simulink model "simulink_slipsl"  (R2022b)
settings: Solver=ode45  StartTime=0.0  StopTime=Tf  FixedStep=1e-3  RelTol=1e-11  AbsTol=1e-11
values from neighbouring files (symbols this model uses):
  flag_dist = [0; 30; 30]    [main.m]    (also in main_slip_w_sw_leg.m = 0)
  gains = [gain.K_p; gain.K_d; gain.K_p_sw; gain.K_d_sw; gain.K_p_ds; gain.K_d_ds; gain.K_v_ds]    [main.m]    (also in main_slip_w_sw_leg.m)
  init_cond = [x_M_init; y_M_init; theta_init; r_init; x_CoM_init; y_CoM_init; dx_M_init; dy_M_init; dtheta_init; dr_init; dx_CoM_init; dy_CoM_init]    [main.m]    (also in main_slip_w_sw_leg.m)
  init_f_record = 0    [main.m]    (also in main_slip_w_sw_leg.m)
  init_flag = [1; dc.col_param.foot; -dc.col_param.footPlus; x_M_init; x_CoM_ss_init; flag_ref_ob]    [main.m]    (also in main_slip_w_sw_leg.m = [1; dc.col_param.foot; -dc.col_param.footPlus; x_M_init; x_C)
  param = [L0_ss; k0_ss; m_M; m_swLeg; m_swFoot; I_swLeg; I_swFoot; L_thigh; k_swFoot; k_swLeg; theta_s0; r_s0; g; L0_ds; k0_ds; bound_cst]    [main.m]    (also in main_slip_w_sw_leg.m = [L0_ss; k0_ss; m_M; m_swLeg; m_swFoot; I_swLeg; I_swFoot; L_)
  ref_star_ds = [ref_star.ds.x_CoM_star,      ref_star.ds.y_CoM_star, ref_star.ds.dx_CoM_star,      ref_star.ds.del_y_CoM_star, ref_star.ds.del_dx_CoM_star,      ref_star.ds.del2_y_CoM_star]    [main.m]    (also in main_slip_w_sw_leg.m)
  ref_star_ss = [ref_star.ss.x_M_star,      ref_star.ss.y_M_star, ref_star.ss.x_swFoot_star, ref_star.ss.y_swFoot_star,      ref_star.ss.del_y_M_star, ref_star.ss.del_x_swFoot_star, ref_star.ss.del_y_swFoot_star,      ref_star.ss.del2_y_M_star, ref_star.ss.del2_x_swFoot_star, ref_star.ss.del2_y_swFoot_star,      ref_star.ss.x_CoM_star]    [main.m]    (also in main_slip_w_sw_leg.m)
  sample_time = 0.001    [main.m]    (also in main_slip_w_sw_leg.m)
libraries: simulink x1
(part 2 of 2)

== matlab function simulink_slipsl/Triggered Subsystem/SLIP-SL controller ==
  data: X input; U output; flag input; ref_star_ss input; ref_star_ds input; gains input; param input; ref_output_ss output; ref_output_ds output; det_A_ss output; det_A_ds output
function [U, ref_output_ss, ref_output_ds, det_A_ss, det_A_ds] = fcn(X, flag, ref_star_ss, ref_star_ds, gains, param)

% ----------- parameters ----------------------
L0_ss = param(1); % [m]
k0_ss = param(2); % nominal leg stiffness [N/m]
m_M = param(3); % hip mass [kg]
m_swLeg = param(4); % [kg]
m_swFoot = param(5); % [kg]
I_swLeg = param(6); %
I_swFoot = param(7); %
L_thigh = param(8); % [m]
k_swFoot = param(9); %
k_swLeg = param(10); %
theta0 = param(11); %[rad]
r0 = param(12); % [m]
gravi = param(13); % gravitational acc

L0_ds = param(14); % [m] free length of the springs in the DS
k0_ds = param(15); % [N/m] stiffness of the springs in the DS

% ----------- flags ----------------------
f_stance = flag(1); % indicates which stance phase it is
foot = flag(2); % location of the stance foot
foot_prev = flag(3) - foot; % previous location of the stance foot
x_M_LO = flag(4); % x_M @LO
x_CoM_LO = flag(5); % x_CoM @LO

% ----------- states ----------------------
x_M = X(1) - foot; % x position of main mass in SS
y_M = X(2); % z position of main mass in SS
theta = X(3); % angle of the swing leg when in SS
r = X(4); % distance of the foot from the knee on SS
x_CoM = X(5) - foot; % x position of the CoM
y_CoM = X(6);

dx_M = X(7); % x velocity of main mass in SS
dy_M = X(8); % z velocity of main mass in SS
dtheta = X(9);
dr = X(10);
dx_CoM = X(11);
dy_CoM = X(12);

q = [x_M; y_M; theta; r; x_CoM; y_CoM];
dq = [dx_M; dy_M; dtheta; dr; dx_CoM; dy_CoM];

%---------- controller -----------------------------

% SS inputs
u1 = 0; % input for stance leg spring
u2 = 0; % input for swing leg torsional spring
u3 = 0; % input for swing foot spring
% DS inputs
u4 = 0; % input for stance leg spring
u5 = 0; % input for swing leg spring

% Controller Gains
K_p = gains(1);
K_d = gains(2);

K_p_sw = gains(3);
K_d_sw = gains(4);

K_p_ds = gains(5);
K_d_ds = gains(6);
K_v_ds = gains(7); % 5 in visser 2012

% for debugging
ref_output_ss = [0; 0; 0];
ref_output_ds = [0;0];
det_A_ss = -1;
det_A_ds = 0;

x_CoM_star_ds = ref_star_ds(:,1);

if f_stance == 1
    % if the system is in single stance phase

    x_CoM_star_ss = ref_star_ss(:,11);

    % updating the x_CoM_star_ss
    x_CoM_des_TD = ref_star_ss(end,11);
    x_CoM_star_ss = x_CoM_star_ss.*((x_CoM_des_TD - x_CoM_LO)/(ref_star_ss(end,11) - ref_star_ss(1,11))) + (x_CoM_LO - ref_star_ss(1,11))/2;

    % calculating x_CoM when for SS phase
    x_swLeg = x_M + (L_thigh/2)*cos(theta);
    x_swFoot = x_M + (L_thigh + r)*cos(theta);
    x_CoM = (m_M*x_M + m_swLeg*x_swLeg + m_swFoot*x_swFoot)/(m_M + m_swLeg + m_swFoot);

    if x_CoM_star_ss(1) <= x_CoM && x_CoM <= x_CoM_star_ss(end)

        % interpolation for references
        y_M_star = interp1(x_CoM_star_ss, ref_star_ss(:,2), x_CoM);
        %         x_swFoot_star = interp1(x_M_star_ss, x_swFoot_ref_mod, x_M);
        x_swFoot_star = interp1(x_CoM_star_ss, ref_star_ss(:,3), x_CoM);
        y_swFoot_star = interp1(x_CoM_star_ss, ref_star_ss(:,4), x_CoM);

        del_y_M_star = interp1(x_CoM_star_ss, ref_star_ss(:,5), x_CoM);
        del_x_swFoot_star = interp1(x_CoM_star_ss, ref_star_ss(:,6), x_CoM);
        del_y_swFoot_star = interp1(x_CoM_star_ss, ref_star_ss(:,7), x_CoM);

        del2_y_M_star = interp1(x_CoM_star_ss, ref_star_ss(:,8), x_CoM);
        del2_x_swFoot_star = interp1(x_CoM_star_ss, ref_star_ss(:,9), x_CoM);
        del2_y_swFoot_star = interp1(x_CoM_star_ss, ref_star_ss(:,10), x_CoM);

        ref_output_ss = [y_M_star; x_swFoot_star; y_swFoot_star];

        % controller

        A_ss = [
            ((L0_ss - (x_M^2 + y_M^2)^(1/2))*(L_thigh^2*m_swLeg^2*y_M + 8*I_swLeg*m_M*y_M + 8*I_swFoot*m_M*y_M + 8*I_swLeg*m_swLeg*y_M + 4*I_swLeg*m_swFoot*y_M + 8*I_swFoot*m_swLeg*y_M + 4*I_swFoot*m_swFoot*y_M + 2*L_thigh^2*m_M*m_swLeg*y_M + 8*L_thigh^2*m_M*m_swFoot*y_M + 5*L_thigh^2*m_swLeg*m_swFoot*y_M + 8*m_M*m_swFoot*r^2*y_M + 8*m_swLeg*m_swFoot*r^2*y_M + L_thigh^2*m_swLeg^2*y_M*cos(2*theta) - L_thigh^2*m_swLeg^2*x_M*sin(2*theta) - 4*I_swLeg*m_swFoot*y_M*cos(2*theta) - 4*I_swFoot*m_swFoot*y_M*cos(2*theta) + 4*I_swLeg*m_swFoot*x_M*sin(2*theta) + 4*I_swFoot*m_swFoot*x_M*sin(2*theta) + 16*L_thigh*m_M*m_swFoot*r*y_M + 12*L_thigh*m_swLeg*m_swFoot*r*y_M + 3*L_thigh^2*m_swLeg*m_swFoot*y_M*cos(2*theta) - 3*L_thigh^2*m_swLeg*m_swFoot*x_M*sin(2*theta) + 4*L_thigh*m_swLeg*m_swFoot*r*y_M*cos(2*theta) - 4*L_thigh*m_swLeg*m_swFoot*r*x_M*sin(2*theta)))/(2*(x_M^2 + y_M^2)^(1/2)*(m_M + m_swLeg)*(4*I_swLeg*m_M + 4*I_swFoot*m_M + 4*I_swLeg*m_swLeg + 4*I_swLeg*m_swFoot + 4*I_swFoot*m_swLeg + 4*I_swFoot*m_swFoot + 4*m_M*m_swFoot*r^2 + 4*m_swLeg*m_swFoot*r^2 + L_thigh^2*m_M*m_swLeg + 4*L_thigh^2*m_M*m_swFoot + L_thigh^2*m_swLeg*m_swFoot + 8*L_thigh*m_M*m_swFoot*r + 4*L_thigh*m_swLeg*m_swFoot*r)) - (del_y_M_star*(L0_ss - (x_M^2 + y_M^2)^(1/2))*((L_thigh^2*m_swLeg^2*x_M)/2 + 4*I_swLeg*m_M*x_M + 4*I_swFoot*m_M*x_M + 4*I_swLeg*m_swLeg*x_M + 2*I_swLeg*m_swFoot*x_M + 4*I_swFoot*m_swLeg*x_M + 2*I_swFoot*m_swFoot*x_M + L_thigh^2*m_M*m_swLeg*x_M + 4*L_thigh^2*m_M*m_swFoot*x_M + (5*L_thigh^2*m_swLeg*m_swFoot*x_M)/2 + 4*m_M*m_swFoot*r^2*x_M + 4*m_swLeg*m_swFoot*r^2*x_M - (L_thigh^2*m_swLeg^2*x_M*cos(2*theta))/2 - (L_thigh^2*m_swLeg^2*y_M*sin(2*theta))/2 + 2*I_swLeg*m_swFoot*x_M*cos(2*theta) + 2*I_swFoot*m_swFoot*x_M*cos(2*theta) + 2*I_swLeg*m_swFoot*y_M*sin(2*theta) + 2*I_swFoot*m_swFoot*y_M*sin(2*theta) + 8*L_thigh*m_M*m_swFoot*r*x_M + 6*L_thigh*m_swLeg*m_swFoot*r*x_M - (3*L_thigh^2*m_swLeg*m_swFoot*x_M*cos(2*theta))/2 - (3*L_thigh^2*m_swLeg*m_swFoot*y_M*sin(2*theta))/2 - 2*L_thigh*m_swLeg*m_swFoot*r*x_M*cos(2*theta) - 2*L_thigh*m_swLeg*m_swFoot*r*y_M*sin(2*theta)))/((x_M^2 + y_M^2)^(1/2)*(m_M + m_swLeg)*(4*I_swLeg*m_M + 4*I_swFoot*m_M + 4*I_swLeg*m_swLeg + 4*I_swLeg*m_swFoot + 4*I_swFoot*m_swLeg + 4*I_swFoot*m_swFoot + 4*m_M*m_swFoot*r^2 + 4*m_swLeg*m_swFoot*r^2 + L_thigh^2*m_M*m_swLeg + 4*L_thigh^2*m_M*m_swFoot + L_thigh^2*m_swLeg*m_swFoot + 8*L_thigh*m_M*m_swFoot*r + 4*L_thigh*m_swLeg*m_swFoot*r)),                                                                                                                                                        (2*(theta - theta0)*(cos(theta) + del_y_M_star*sin(theta))*(L_thigh*m_swLeg + 2*L_thigh*m_swFoot + 2*m_swFoot*r))/(4*I_swLeg*m_M + 4*I_swFoot*m_M + 4*I_swLeg*m_swLeg + 4*I_swLeg*m_swFoot + 4*I_swFoot*m_swLeg + 4*I_swFoot*m_swFoot + 4*m_M*m_swFoot*r^2 + 4*m_swLeg*m_swFoot*r^2 + L_thigh^2*m_M*m_swLeg + 4*L_thigh^2*m_M*m_swFoot + L_thigh^2*m_swLeg*m_swFoot + 8*L_thigh*m_M*m_swFoot*r + 4*L_thigh*m_swLeg*m_swFoot*r),                                                    ((r - r0)*(sin(theta) - del_y_M_star*cos(theta)))/(m_M + m_swLeg)
            (2*sin(theta)*(L_thigh + r)*(L0_ss - (x_M^2 + y_M^2)^(1/2))*(y_M*cos(theta) - x_M*sin(theta))*(L_thigh*m_swLeg + 2*L_thigh*m_swFoot + 2*m_swFoot*r))/((x_M^2 + y_M^2)^(1/2)*(4*I_swLeg*m_M + 4*I_swFoot*m_M + 4*I_swLeg*m_swLeg + 4*I_swLeg*m_swFoot + 4*I_swFoot*m_swLeg + 4*I_swFoot*m_swFoot + 4*m_M*m_swFoot*r^2 + 4*m_swLeg*m_swFoot*r^2 + L_thigh^2*m_M*m_swLeg + 4*L_thigh^2*m_M*m_swFoot + L_thigh^2*m_swLeg*m_swFoot + 8*L_thigh*m_M*m_swFoot*r + 4*L_thigh*m_swLeg*m_swFoot*r)) - ((L0_ss - (x_M^2 + y_M^2)^(1/2))*(del_x_swFoot_star - 1)*((L_thigh^2*m_swLeg^2*x_M)/2 + 4*I_swLeg*m_M*x_M + 4*I_swFoot*m_M*x_M + 4*I_swLeg*m_swLeg*x_M + 2*I_swLeg*m_swFoot*x_M + 4*I_swFoot*m_swLeg*x_M + 2*I_swFoot*m_swFoot*x_M + L_thigh^2*m_M*m_swLeg*x_M + 4*L_thigh^2*m_M*m_swFoot*x_M + (5*L_thigh^2*m_swLeg*m_swFoot*x_M)/2 + 4*m_M*m_swFoot*r^2*x_M + 4*m_swLeg*m_swFoot*r^2*x_M - (L_thigh^2*m_swLeg^2*x_M*cos(2*theta))/2 - (L_thigh^2*m_swLeg^2*y_M*sin(2*theta))/2 + 2*I_swLeg*m_swFoot*x_M*cos(2*theta) + 2*I_swFoot*m_swFoot*x_M*cos(2*theta) + 2*I_swLeg*m_swFoot*y_M*sin(2*theta) + 2*I_swFoot*m_swFoot*y_M*sin(2*theta) + 8*L_thigh*m_M*m_swFoot*r*x_M + 6*L_thigh*m_swLeg*m_swFoot*r*x_M - (3*L_thigh^2*m_swLeg*m_swFoot*x_M*cos(2*theta))/2 - (3*L_thigh^2*m_swLeg*m_swFoot*y_M*sin(2*theta))/2 - 2*L_thigh*m_swLeg*m_swFoot*r*x_M*cos(2*theta) - 2*L_thigh*m_swLeg*m_swFoot*r*y_M*sin(2*theta)))/((x_M^2 + y_M^2)^(1/2)*(m_M + m_swLeg)*(4*I_swLeg*m_M + 4*I_swFoot*m_M + 4*I_swLeg*m_swLeg + 4*I_swLeg*m_swFoot + 4*I_swFoot*m_swLeg + 4*I_swFoot*m_swFoot + 4*m_M*m_swFoot*r^2 + 4*m_swLeg*m_swFoot*r^2 + L_thigh^2*m_M*m_swLeg + 4*L_thigh^2*m_M*m_swFoot + L_thigh^2*m_swLeg*m_swFoot + 8*L_thigh*m_M*m_swFoot*r + 4*L_thigh*m_swLeg*m_swFoot*r)) - (cos(theta)*(L0_ss - (x_M^2 + y_M^2)^(1/2))*(x_M*cos(theta) + y_M*sin(theta)))/((x_M^2 + y_M^2)^(1/2)*(m_M + m_swLeg)),                                                                    (2*sin(theta)*(theta - theta0)*(2*L_thigh*m_M + L_thigh*m_swLeg + 2*m_M*r + 2*m_swLeg*r + L_thigh*del_x_swFoot_star*m_swLeg + 2*L_thigh*del_x_swFoot_star*m_swFoot + 2*del_x_swFoot_star*m_swFoot*r))/(4*I_swLeg*m_M + 4*I_swFoot*m_M + 4*I_swLeg*m_swLeg + 4*I_swLeg*m_swFoot + 4*I_swFoot*m_swLeg + 4*I_swFoot*m_swFoot + 4*m_M*m_swFoot*r^2 + 4*m_swLeg*m_swFoot*r^2 + L_thigh^2*m_M*m_swLeg + 4*L_thigh^2*m_M*m_swFoot + L_thigh^2*m_swLeg*m_swFoot + 8*L_thigh*m_M*m_swFoot*r + 4*L_thigh*m_swLeg*m_swFoot*r),                       -(cos(theta)*(r - r0)*(m_M + m_swLeg + del_x_swFoot_star*m_swFoot))/(m_swFoot*(m_M + m_swLeg))
            ((L0_ss - (x_M^2 + y_M^2)^(1/2))*(L_thigh^2*m_swLeg^2*y_M + 8*I_swLeg*m_M*y_M + 8*I_swFoot*m_M*y_M + 8*I_swLeg*m_swLeg*y_M + 4*I_swLeg*m_swFoot*y_M + 8*I_swFoot*m_swLeg*y_M + 4*I_swFoot*m_swFoot*y_M + 2*L_thigh^2*m_M*m_swLeg*y_M + 8*L_thigh^2*m_M*m_swFoot*y_M + 5*L_thigh^2*m_swLeg*m_swFoot*y_M + 8*m_M*m_swFoot*r^2*y_M + 8*m_swLeg*m_swFoot*r^2*y_M + L_thigh^2*m_swLeg^2*y_M*cos(2*theta) - L_thigh^2*m_swLeg^2*x_M*sin(2*theta) - 4*I_swLeg*m_swFoot*y_M*cos(2*theta) - 4*I_swFoot*m_swFoot*y_M*cos(2*theta) + 4*I_swLeg*m_swFoot*x_M*sin(2*theta) + 4*I_swFoot*m_swFoot*x_M*sin(2*theta) + 16*L_thigh*m_M*m_swFoot*r*y_M + 12*L_thigh*m_swLeg*m_swFoot*r*y_M + 3*L_thigh^2*m_swLeg*m_swFoot*y_M*cos(2*theta) - 3*L_thigh^2*m_swLeg*m_swFoot*x_M*sin(2*theta) + 4*L_thigh*m_swLeg*m_swFoot*r*y_M*cos(2*theta) - 4*L_thigh*m_swLeg*m_swFoot*r*x_M*sin(2*theta)))/(2*(x_M^2 + y_M^2)^(1/2)*(m_M + m_swLeg)*(4*I_swLeg*m_M + 4*I_swFoot*m_M + 4*I_swLeg*m_swLeg + 4*I_swLeg*m_swFoot + 4*I_swFoot*m_swLeg + 4*I_swFoot*m_swFoot + 4*m_M*m_swFoot*r^2 + 4*m_swLeg*m_swFoot*r^2 + L_thigh^2*m_M*m_swLeg + 4*L_thigh^2*m_M*m_swFoot + L_thigh^2*m_swLeg*m_swFoot + 8*L_thigh*m_M*m_swFoot*r + 4*L_thigh*m_swLeg*m_swFoot*r)) - (sin(theta)*(L0_ss - (x_M^2 + y_M^2)^(1/2))*(x_M*cos(theta) + y_M*sin(theta)))/((x_M^2 + y_M^2)^(1/2)*(m_M + m_swLeg)) - (del_y_swFoot_star*(L0_ss - (x_M^2 + y_M^2)^(1/2))*((L_thigh^2*m_swLeg^2*x_M)/2 + 4*I_swLeg*m_M*x_M + 4*I_swFoot*m_M*x_M + 4*I_swLeg*m_swLeg*x_M + 2*I_swLeg*m_swFoot*x_M + 4*I_swFoot*m_swLeg*x_M + 2*I_swFoot*m_swFoot*x_M + L_thigh^2*m_M*m_swLeg*x_M + 4*L_thigh^2*m_M*m_swFoot*x_M + (5*L_thigh^2*m_swLeg*m_swFoot*x_M)/2 + 4*m_M*m_swFoot*r^2*x_M + 4*m_swLeg*m_swFoot*r^2*x_M - (L_thigh^2*m_swLeg^2*x_M*cos(2*theta))/2 - (L_thigh^2*m_swLeg^2*y_M*sin(2*theta))/2 + 2*I_swLeg*m_swFoot*x_M*cos(2*theta) + 2*I_swFoot*m_swFoot*x_M*cos(2*theta) + 2*I_swLeg*m_swFoot*y_M*sin(2*theta) + 2*I_swFoot*m_swFoot*y_M*sin(2*theta) + 8*L_thigh*m_M*m_swFoot*r*x_M + 6*L_thigh*m_swLeg*m_swFoot*r*x_M - (3*L_thigh^2*m_swLeg*m_swFoot*x_M*cos(2*theta))/2 - (3*L_thigh^2*m_swLeg*m_swFoot*y_M*sin(2*theta))/2 - 2*L_thigh*m_swLeg*m_swFoot*r*x_M*cos(2*theta) - 2*L_thigh*m_swLeg*m_swFoot*r*y_M*sin(2*theta)))/((x_M^2 + y_M^2)^(1/2)*(m_M + m_swLeg)*(4*I_swLeg*m_M + 4*I_swFoot*m_M + 4*I_swLeg*m_swLeg + 4*I_swLeg*m_swFoot + 4*I_swFoot*m_swLeg + 4*I_swFoot*m_swFoot + 4*m_M*m_swFoot*r^2 + 4*m_swLeg*m_swFoot*r^2 + L_thigh^2*m_M*m_swLeg + 4*L_thigh^2*m_M*m_swFoot + L_thigh^2*m_swLeg*m_swFoot + 8*L_thigh*m_M*m_swFoot*r + 4*L_thigh*m_swLeg*m_swFoot*r)) - (2*cos(theta)*(L_thigh + r)*(L0_ss - (x_M^2 + y_M^2)^(1/2))*(y_M*cos(theta) - x_M*sin(theta))*(L_thigh*m_swLeg + 2*L_thigh*m_swFoot + 2*m_swFoot*r))/((x_M^2 + y_M^2)^(1/2)*(4*I_swLeg*m_M + 4*I_swFoot*m_M + 4*I_swLeg*m_swLeg + 4*I_swLeg*m_swFoot + 4*I_swFoot*m_swLeg + 4*I_swFoot*m_swFoot + 4*m_M*m_swFoot*r^2 + 4*m_swLeg*m_swFoot*r^2 + L_thigh^2*m_M*m_swLeg + 4*L_thigh^2*m_M*m_swFoot + L_thigh^2*m_swLeg*m_swFoot + 8*L_thigh*m_M*m_swFoot*r + 4*L_thigh*m_swLeg*m_swFoot*r)), -(2*(theta - theta0)*(2*m_M*r*cos(theta) + 2*m_swLeg*r*cos(theta) + 2*L_thigh*m_M*cos(theta) + L_thigh*m_swLeg*cos(theta) - L_thigh*del_y_swFoot_star*m_swLeg*sin(theta) - 2*L_thigh*del_y_swFoot_star*m_swFoot*sin(theta) - 2*del_y_swFoot_star*m_swFoot*r*sin(theta)))/(4*I_swLeg*m_M + 4*I_swFoot*m_M + 4*I_swLeg*m_swLeg + 4*I_swLeg*m_swFoot + 4*I_swFoot*m_swLeg + 4*I_swFoot*m_swFoot + 4*m_M*m_swFoot*r^2 + 4*m_swLeg*m_swFoot*r^2 + L_thigh^2*m_M*m_swLeg + 4*L_thigh^2*m_M*m_swFoot + L_thigh^2*m_swLeg*m_swFoot + 8*L_thigh*m_M*m_swFoot*r + 4*L_thigh*m_swLeg*m_swFoot*r), -((r - r0)*(m_M*sin(theta) + m_swLeg*sin(theta) + del_y_swFoot_star*m_swFoot*cos(theta)))/(m_swFoot*(m_M + m_swLeg))];

        K_ss = [
            del2_y_M_star*dx_M^2 - K_p*(y_M - y_M_star) - K_d*(dy_M - del_y_M_star*dx_M) + (8*I_swLeg*gravi*m_M^2*(x_M^2 + y_M^2)^(1/2) + 8*I_swFoot*gravi*m_M^2*(x_M^2 + y_M^2)^(1/2) + 8*I_swLeg*gravi*m_swLeg^2*(x_M^2 + y_M^2)^(1/2) + 8*I_swFoot*gravi*m_swLeg^2*(x_M^2 + y_M^2)^(1/2) - L0_ss*L_thigh^2*k0_ss*m_swLeg^2*y_M + 2*L_thigh^2*gravi*m_M*m_swLeg^2*(x_M^2 + y_M^2)^(1/2) + 2*L_thigh^2*gravi*m_M^2*m_swLeg*(x_M^2 + y_M^2)^(1/2) + 8*L_thigh^2*gravi*m_M^2*m_swFoot*(x_M^2 + y_M^2)^(1/2) + 2*L_thigh^2*gravi*m_swLeg^2*m_swFoot*(x_M^2 + y_M^2)^(1/2) + L_thigh^2*k0_ss*m_swLeg^2*y_M*(x_M^2 + y_M^2)^(1/2) + 8*gravi*m_M^2*m_swFoot*r^2*(x_M^2 + y_M^2)^(1/2) + 8*gravi*m_swLeg^2*m_swFoot*r^2*(x_M^2 + y_M^2)^(1/2) - 8*I_swLeg*L0_ss*k0_ss*m_M*y_M - 8*I_swFoot*L0_ss*k0_ss*m_M*y_M - 8*I_swLeg*L0_ss*k0_ss*m_swLeg*y_M - 4*I_swLeg*L0_ss*k0_ss*m_swFoot*y_M - 8*I_swFoot*L0_ss*k0_ss*m_swLeg*y_M - 4*I_swFoot*L0_ss*k0_ss*m_swFoot*y_M + 16*I_swLeg*gravi*m_M*m_swLeg*(x_M^2 + y_M^2)^(1/2) + 8*I_swLeg*gravi*m_M*m_swFoot*(x_M^2 + y_M^2)^(1/2) + 16*I_swFoot*gravi*m_M*m_swLeg*(x_M^2 + y_M^2)^(1/2) + 8*I_swFoot*gravi*m_M*m_swFoot*(x_M^2 + y_M^2)^(1/2) + 8*I_swLeg*gravi*m_swLeg*m_swFoot*(x_M^2 + y_M^2)^(1/2) + 8*I_swFoot*gravi*m_swLeg*m_swFoot*(x_M^2 + y_M^2)^(1/2) + 8*I_swLeg*k0_ss*m_M*y_M*(x_M^2 + y_M^2)^(1/2) + 8*I_swFoot*k0_ss*m_M*y_M*(x_M^2 + y_M^2)^(1/2) + 8*I_swLeg*k0_ss*m_swLeg*y_M*(x_M^2 + y_M^2)^(1/2) + 4*I_swLeg*k0_ss*m_swFoot*y_M*(x_M^2 + y_M^2)^(1/2) + 8*I_swFoot*k0_ss*m_swLeg*y_M*(x_M^2 + y_M^2)^(1/2) + 4*I_swFoot*k0_ss*m_swFoot*y_M*(x_M^2 + y_M^2)^(1/2) - 2*L0_ss*L_thigh^2*k0_ss*m_M*m_swLeg*y_M - 8*L0_ss*L_thigh^2*k0_ss*m_M*m_swFoot*y_M - 5*L0_ss*L_thigh^2*k0_ss*m_swLeg*m_swFoot*y_M + 10*L_thigh^2*gravi*m_M*m_swLeg*m_swFoot*(x_M^2 + y_M^2)^(1/2) + 16*L_thigh*gravi*m_M^2*m_swFoot*r*(x_M^2 + y_M^2)^(1/2) + 8*L_thigh*gravi*m_swLeg^2*m_swFoot*r*(x_M^2 + y_M^2)^(1/2) + 2*L_thigh^2*k0_ss*m_M*m_swLeg*y_M*(x_M^2 + y_M^2)^(1/2) + 8*L_thigh^2*k0_ss*m_M*m_swFoot*y_M*(x_M^2 + y_M^2)^(1/2) + 5*L_thigh^2*k0_ss*m_swLeg*m_swFoot*y_M*(x_M^2 + y_M^2)^(1/2) - 8*L0_ss*k0_ss*m_M*m_swFoot*r^2*y_M - 8*L0_ss*k0_ss*m_swLeg*m_swFoot*r^2*y_M - L0_ss*L_thigh^2*k0_ss*m_swLeg^2*y_M*cos(2*theta) - 8*I_swLeg*k_swFoot*m_M*r*sin(theta)*(x_M^2 + y_M^2)^(1/2) + 8*I_swLeg*k_swFoot*m_M*r0*sin(theta)*(x_M^2 + y_M^2)^(1/2) - 8*I_swFoot*k_swFoot*m_M*r*sin(theta)*(x_M^2 + y_M^2)^(1/2) + 8*I_swFoot*k_swFoot*m_M*r0*sin(theta)*(x_M^2 + y_M^2)^(1/2) - 8*I_swLeg*k_swFoot*m_swLeg*r*sin(theta)*(x_M^2 + y_M^2)^(1/2) + 8*I_swLeg*k_swFoot*m_swLeg*r0*sin(theta)*(x_M^2 + y_M^2)^(1/2) - 8*I_swLeg*k_swFoot*m_swFoot*r*sin(theta)*(x_M^2 + y_M^2)^(1/2) + 8*I_swLeg*k_swFoot*m_swFoot*r0*sin(theta)*(x_M^2 + y_M^2)^(1/2) - 8*I_swFoot*k_swFoot*m_swLeg*r*sin(theta)*(x_M^2 + y_M^2)^(1/2) + 8*I_swFoot*k_swFoot*m_swLeg*r0*sin(theta)*(x_M^2 + y_M^2)^(1/2) - 8*I_swFoot*k_swFoot*m_swFoot*r*sin(theta)*(x_M^2 + y_M^2)^(1/2) + 8*I_swFoot*k_swFoot*m_swFoot*r0*sin(theta)*(x_M^2 + y_M^2)^(1/2) + L0_ss*L_thigh^2*k0_ss*m_swLeg^2*x_M*sin(2*theta) + 16*gravi*m_M*m_swLeg*m_swFoot*r^2*(x_M^2 + y_M^2)^(1/2) + 8*k0_ss*m_M*m_swFoot*r^2*y_M*(x_M^2 + y_M^2)^(1/2) + 8*k0_ss*m_swLeg*m_swFoot*r^2*y_M*(x_M^2 + y_M^2)^(1/2) - L_thigh^3*dtheta^2*m_M*m_swLeg^2*sin(theta)*(x_M^2 + y_M^2)^(1/2) - L_thigh^3*dtheta^2*m_swLeg^2*m_swFoot*sin(theta)*(x_M^2 + y_M^2)^(1/2) + L_thigh^2*k0_ss*m_swLeg^2*y_M*cos(2*theta)*(x_M^2 + y_M^2)^(1/2) - L_thigh^2*k0_ss*m_swLeg^2*x_M*sin(2*theta)*(x_M^2 + y_M^2)^(1/2) + 4*I_swLeg*L0_ss*k0_ss*m_swFoot*y_M*cos(2*theta) + 4*I_swFoot*L0_ss*k0_ss*m_swFoot*y_M*cos(2*theta) - 4*I_swLeg*L0_ss*k0_ss*m_swFoot*x_M*sin(2*theta) - 4*I_swFoot*L0_ss*k0_ss*m_swFoot*x_M*sin(2*theta) - 4*L_thigh*k_swLeg*m_swLeg^2*theta*cos(theta)*(x_M^2 + y_M^2)^(1/2) + 4*L_thigh*k_swLeg*m_swLeg^2*theta0*cos(theta)*(x_M^2 + y_M^2)^(1/2) - 4*I_swLeg*k0_ss*m_swFoot*y_M*cos(2*theta)*(x_M^2 + y_M^2)^(1/2) - 4*I_swFoot*k0_ss*m_swFoot*y_M*cos(2*theta)*(x_M^2 + y_M^2)^(1/2) + 4*I_swLeg*k0_ss*m_swFoot*x_M*sin(2*theta)*(x_M^2 + y_M^2)^(1/2) + 4*I_swFoot*k0_ss*m_swFoot*x_M*sin(2*theta)*(x_M^2 + y_M^2)^(1/2) - 8*k_swFoot*m_M*m_swFoot*r^3*sin(theta)*(x_M^2 + y_M^2)^(1/2) - 8*k_swFoot*m_swLeg*m_swFoot*r^3*sin(theta)*(x_M^2 + y_M^2)^(1/2) - 4*I_swLeg*L_thigh*dtheta^2*m_swLeg^2*sin(theta)*(x_M^2 + y_M^2)^(1/2) - 4*I_swFoot*L_thigh*dtheta^2*m_swLeg^2*sin(theta)*(x_M^2 + y_M^2)^(1/2) - 2*L_thigh^2*k_swFoot*m_M*m_swLeg*r*sin(theta)*(x_M^2 + y_M^2)^(1/2) + 2*L_thigh^2*k_swFoot*m_M*m_swLeg*r0*sin(theta)*(x_M^2 + y_M^2)^(1/2) - 16*L_thigh*k_swFoot*m_M*m_swFoot*r^2*sin(theta)*(x_M^2 + y_M^2)^(1/2) - 8*L_thigh^2*k_swFoot*m_M*m_swFoot*r*sin(theta)*(x_M^2 + y_M^2)^(1/2) + 8*L_thigh^2*k_swFoot*m_M*m_swFoot*r0*sin(theta)*(x_M^2 + y_M^2)^(1/2) - 8*L_thigh*k_swFoot*m_swLeg*m_swFoot*r^2*sin(theta)*(x_M^2 + y_M^2)^(1/2) - 2*L_thigh^2*k_swFoot*m_swLeg*m_swFoot*r*sin(theta)*(x_M^2 + y_M^2)^(1/2) + 2*L_thigh^2*k_swFoot*m_swLeg*m_swFoot*r0*sin(theta)*(x_M^2 + y_M^2)^(1/2) - 16*L0_ss*L_thigh*k0_ss*m_M*m_swFoot*r*y_M - 12*L0_ss*L_thigh*k0_ss*m_swLeg*m_swFoot*r*y_M + 24*L_thigh*gravi*m_M*m_swLeg*m_swFoot*r*(x_M^2 + y_M^2)^(1/2) + 8*k_swFoot*m_M*m_swFoot*r^2*r0*sin(theta)*(x_M^2 + y_M^2)^(1/2) + 8*k_swFoot*m_swLeg*m_swFoot*r^2*r0*sin(theta)*(x_M^2 + y_M^2)^(1/2) + 16*L_thigh*k0_ss*m_M*m_swFoot*r*y_M*(x_M^2 + y_M^2)^(1/2) + 12*L_thigh*k0_ss*m_swLeg*m_swFoot*r*y_M*(x_M^2 + y_M^2)^(1/2) - 3*L0_ss*L_thigh^2*k0_ss*m_swLeg*m_swFoot*y_M*cos(2*theta) - 4*L_thigh^2*dr*dtheta*m_swLeg^2*m_swFoot*cos(theta)*(x_M^2 + y_M^2)^(1/2) + 3*L0_ss*L_thigh^2*k0_ss*m_swLeg*m_swFoot*x_M*sin(2*theta) - 4*L_thigh^3*dtheta^2*m_M*m_swLeg*m_swFoot*sin(theta)*(x_M^2 + y_M^2)^(1/2) + 3*L_thigh^2*k0_ss*m_swLeg*m_swFoot*y_M*cos(2*theta)*(x_M^2 + y_M^2)^(1/2) - 3*L_thigh^2*k0_ss*m_swLeg*m_swFoot*x_M*sin(2*theta)*(x_M^2 + y_M^2)^(1/2) + 16*I_swLeg*dr*dtheta*m_M*m_swFoot*cos(theta)*(x_M^2 + y_M^2)^(1/2) + 16*I_swFoot*dr*dtheta*m_M*m_swFoot*cos(theta)*(x_M^2 + y_M^2)^(1/2) + 16*I_swLeg*dr*dtheta*m_swLeg*m_swFoot*cos(theta)*(x_M^2 + y_M^2)^(1/2) + 16*I_swFoot*dr*dtheta*m_swLeg*m_swFoot*cos(theta)*(x_M^2 + y_M^2)^(1/2) - 4*L_thigh*k_swLeg*m_M*m_swLeg*theta*cos(theta)*(x_M^2 + y_M^2)^(1/2) + 4*L_thigh*k_swLeg*m_M*m_swLeg*theta0*cos(theta)*(x_M^2 + y_M^2)^(1/2) - 8*L_thigh*k_swLeg*m_M*m_swFoot*theta*cos(theta)*(x_M^2 + y_M^2)^(1/2) + 8*L_thigh*k_swLeg*m_M*m_swFoot*theta0*cos(theta)*(x_M^2 + y_M^2)^(1/2) - 8*L_thigh*k_swLeg*m_swLeg*m_swFoot*theta*cos(theta)*(x_M^2 + y_M^2)^(1/2) + 8*L_thigh*k_swLeg*m_swLeg*m_swFoot*theta0*cos(theta)*(x_M^2 + y_M^2)^(1/2) - 4*L_thigh*dtheta^2*m_swLeg^2*m_swFoot*r^2*sin(theta)*(x_M^2 + y_M^2)^(1/2) - 4*L_thigh^2*dtheta^2*m_swLeg^2*m_swFoot*r*sin(theta)*(x_M^2 + y_M^2)^(1/2) - 8*k_swLeg*m_M*m_swFoot*r*theta*cos(theta)*(x_M^2 + y_M^2)^(1/2) + 8*k_swLeg*m_M*m_swFoot*r*theta0*cos(theta)*(x_M^2 + y_M^2)^(1/2) - 8*k_swLeg*m_swLeg*m_swFoot*r*theta*cos(theta)*(x_M^2 + y_M^2)^(1/2) + 8*k_swLeg*m_swLeg*m_swFoot*r*theta0*cos(theta)*(x_M^2 + y_M^2)^(1/2) - 4*I_swLeg*L_thigh*dtheta^2*m_M*m_swLeg*sin(theta)*(x_M^2 + y_M^2)^(1/2) - 4*I_swFoot*L_thigh*dtheta^2*m_M*m_swLeg*sin(theta)*(x_M^2 + y_M^2)^(1/2) - 4*I_swLeg*L_thigh*dtheta^2*m_swLeg*m_swFoot*sin(theta)*(x_M^2 + y_M^2)^(1/2) - 4*I_swFoot*L_thigh*dtheta^2*m_swLeg*m_swFoot*sin(theta)*(x_M^2 + y_M^2)^(1/2) + 16*L_thigh*k_swFoot*m_M*m_swFoot*r*r0*sin(theta)*(x_M^2 + y_M^2)^(1/2) + 8*L_thigh*k_swFoot*m_swLeg*m_swFoot*r*r0*sin(theta)*(x_M^2 + y_M^2)^(1/2) - 4*L0_ss*L_thigh*k0_ss*m_swLeg*m_swFoot*r*y_M*cos(2*theta) - 4*L_thigh^2*dr*dtheta*m_M*m_swLeg*m_swFoot*cos(theta)*(x_M^2 + y_M^2)^(1/2) - 8*L_thigh*dr*dtheta*m_swLeg^2*m_swFoot*r*cos(theta)*(x_M^2 + y_M^2)^(1/2) + 4*L0_ss*L_thigh*k0_ss*m_swLeg*m_swFoot*r*x_M*sin(2*theta) + 4*L_thigh*k0_ss*m_swLeg*m_swFoot*r*y_M*cos(2*theta)*(x_M^2 + y_M^2)^(1/2) - 4*L_thigh*k0_ss*m_swLeg*m_swFoot*r*x_M*sin(2*theta)*(x_M^2 + y_M^2)^(1/2) - 4*L_thigh*dtheta^2*m_M*m_swLeg*m_swFoot*r^2*sin(theta)*(x_M^2 + y_M^2)^(1/2) - 8*L_thigh^2*dtheta^2*m_M*m_swLeg*m_swFoot*r*sin(theta)*(x_M^2 + y_M^2)^(1/2) - 8*L_thigh*dr*dtheta*m_M*m_swLeg*m_swFoot*r*cos(theta)*(x_M^2 + y_M^2)^(1/2))/(2*(x_M^2 + y_M^2)^(1/2)*(m_M + m_swLeg)*(4*I_swLeg*m_M + 4*I_swFoot*m_M + 4*I_swLeg*m_swLeg + 4*I_swLeg*m_swFoot + 4*I_swFoot*m_swLeg + 4*I_swFoot*m_swFoot + 4*m_M*m_swFoot*r^2 + 4*m_swLeg*m_swFoot*r^2 + L_thigh^2*m_M*m_swLeg + 4*L_thigh^2*m_M*m_swFoot + L_thigh^2*m_swLeg*m_swFoot + 8*L_thigh*m_M*m_swFoot*r + 4*L_thigh*m_swLeg*m_swFoot*r)) + (del_y_M_star*(2*L0_ss*L_thigh^2*k0_ss*m_swLeg^2*x_M - 2*L_thigh^2*k0_ss*m_swLeg^2*x_M*(x_M^2 + y_M^2)^(1/2) + 8*I_swLeg*L0_ss*k0_ss*m_M*x_M + 8*I_swFoot*L0_ss*k0_ss*m_M*x_M + 8*I_swLeg*L0_ss*k0_ss*m_swLeg*x_M + 8*I_swFoot*L0_ss*k0_ss*m_swLeg*x_M - 8*I_swLeg*k0_ss*m_M*x_M*(x_M^2 + y_M^2)^(1/2) - 8*I_swFoot*k0_ss*m_M*x_M*(x_M^2 + y_M^2)^(1/2) - 8*I_swLeg*k0_ss*m_swLeg*x_M*(x_M^2 + y_M^2)^(1/2) - 8*I_swFoot*k0_ss*m_swLeg*x_M*(x_M^2 + y_M^2)^(1/2) + 2*L0_ss*L_thigh^2*k0_ss*m_M*m_swLeg*x_M + 8*L0_ss*L_thigh^2*k0_ss*m_M*m_swFoot*x_M + 8*L0_ss*L_thigh^2*k0_ss*m_swLeg*m_swFoot*x_M - 2*L_thigh^2*k0_ss*m_M*m_swLeg*x_M*(x_M^2 + y_M^2)^(1/2) - 8*L_thigh^2*k0_ss*m_M*m_swFoot*x_M*(x_M^2 + y_M^2)^(1/2) - 8*L_thigh^2*k0_ss*m_swLeg*m_swFoot*x_M*(x_M^2 + y_M^2)^(1/2) + 8*I_swLeg*k_swFoot*m_M*r*cos(theta)*(x_M^2 + y_M^2)^(1/2) - 8*I_swLeg*k_swFoot*m_M*r0*cos(theta)*(x_M^2 + y_M^2)^(1/2) + 8*I_swFoot*k_swFoot*m_M*r*cos(theta)*(x_M^2 + y_M^2)^(1/2) - 8*I_swFoot*k_swFoot*m_M*r0*cos(theta)*(x_M^2 + y_M^2)^(1/2) + 8*I_swLeg*k_swFoot*m_swLeg*r*cos(theta)*(x_M^2 + y_M^2)^(1/2) - 8*I_swLeg*k_swFoot*m_swLeg*r0*cos(theta)*(x_M^2 + y_M^2)^(1/2) + 8*I_swLeg*k_swFoot*m_swFoot*r*cos(theta)*(x_M^2 + y_M^2)^(1/2) - 8*I_swLeg*k_swFoot*m_swFoot*r0*cos(theta)*(x_M^2 + y_M^2)^(1/2) + 8*I_swFoot*k_swFoot*m_swLeg*r*cos(theta)*(x_M^2 + y_M^2)^(1/2) - 8*I_swFoot*k_swFoot*m_swLeg*r0*cos(theta)*(x_M^2 + y_M^2)^(1/2) + 8*I_swFoot*k_swFoot*m_swFoot*r*cos(theta)*(x_M^2 + y_M^2)^(1/2) - 8*I_swFoot*k_swFoot*m_swFoot*r0*cos(theta)*(x_M^2 + y_M^2)^(1/2) + 8*L0_ss*k0_ss*m_M*m_swFoot*r^2*x_M + 8*L0_ss*k0_ss*m_swLeg*m_swFoot*r^2*x_M - 2*L0_ss*L_thigh^2*k0_ss*m_swLeg^2*x_M*cos(theta)^2 - L0_ss*L_thigh^2*k0_ss*m_swLeg^2*y_M*sin(2*theta) + L_thigh^3*dtheta^2*m_M*m_swLeg^2*cos(theta)*(x_M^2 + y_M^2)^(1/2) + L_thigh^3*dtheta^2*m_swLeg^2*m_swFoot*cos(theta)*(x_M^2 + y_M^2)^(1/2) - 8*k0_ss*m_M*m_swFoot*r^2*x_M*(x_M^2 + y_M^2)^(1/2) - 8*k0_ss*m_swLeg*m_swFoot*r^2*x_M*(x_M^2 + y_M^2)^(1/2) + 2*L_thigh^2*k0_ss*m_swLeg^2*x_M*cos(theta)^2*(x_M^2 + y_M^2)^(1/2) + L_thigh^2*k0_ss*m_swLeg^2*y_M*sin(2*theta)*(x_M^2 + y_M^2)^(1/2) + 8*I_swLeg*L0_ss*k0_ss*m_swFoot*x_M*cos(theta)^2 + 8*I_swFoot*L0_ss*k0_ss*m_swFoot*x_M*cos(theta)^2 + 4*I_swLeg*L0_ss*k0_ss*m_swFoot*y_M*sin(2*theta) + 4*I_swFoot*L0_ss*k0_ss*m_swFoot*y_M*sin(2*theta) - 8*I_swLeg*k0_ss*m_swFoot*x_M*cos(theta)^2*(x_M^2 + y_M^2)^(1/2) - 8*I_swFoot*k0_ss*m_swFoot*x_M*cos(theta)^2*(x_M^2 + y_M^2)^(1/2) - 4*L_thigh*k_swLeg*m_swLeg^2*theta*sin(theta)*(x_M^2 + y_M^2)^(1/2) + 4*L_thigh*k_swLeg*m_swLeg^2*theta0*sin(theta)*(x_M^2 + y_M^2)^(1/2) - 4*I_swLeg*k0_ss*m_swFoot*y_M*sin(2*theta)*(x_M^2 + y_M^2)^(1/2) - 4*I_swFoot*k0_ss*m_swFoot*y_M*sin(2*theta)*(x_M^2 + y_M^2)^(1/2) + 8*k_swFoot*m_M*m_swFoot*r^3*cos(theta)*(x_M^2 + y_M^2)^(1/2) + 8*k_swFoot*m_swLeg*m_swFoot*r^3*cos(theta)*(x_M^2 + y_M^2)^(1/2) + 4*I_swLeg*L_thigh*dtheta^2*m_swLeg^2*cos(theta)*(x_M^2 + y_M^2)^(1/2) + 4*I_swFoot*L_thigh*dtheta^2*m_swLeg^2*cos(theta)*(x_M^2 + y_M^2)^(1/2) + 2*L_thigh^2*k_swFoot*m_M*m_swLeg*r*cos(theta)*(x_M^2 + y_M^2)^(1/2) - 2*L_thigh^2*k_swFoot*m_M*m_swLeg*r0*cos(theta)*(x_M^2 + y_M^2)^(1/2) + 16*L_thigh*k_swFoot*m_M*m_swFoot*r^2*cos(theta)*(x_M^2 + y_M^2)^(1/2) + 8*L_thigh^2*k_swFoot*m_M*m_swFoot*r*cos(theta)*(x_M^2 + y_M^2)^(1/2) - 8*L_thigh^2*k_swFoot*m_M*m_swFoot*r0*cos(theta)*(x_M^2 + y_M^2)^(1/2) + 8*L_thigh*k_swFoot*m_swLeg*m_swFoot*r^2*cos(theta)*(x_M^2 + y_M^2)^(1/2) + 2*L_thigh^2*k_swFoot*m_swLeg*m_swFoot*r*cos(theta)*(x_M^2 + y_M^2)^(1/2) - 2*L_thigh^2*k_swFoot*m_swLeg*m_swFoot*r0*cos(theta)*(x_M^2 + y_M^2)^(1/2) + 16*L0_ss*L_thigh*k0_ss*m_M*m_swFoot*r*x_M + 16*L0_ss*L_thigh*k0_ss*m_swLeg*m_swFoot*r*x_M - 8*k_swFoot*m_M*m_swFoot*r^2*r0*cos(theta)*(x_M^2 + y_M^2)^(1/2) - 8*k_swFoot*m_swLeg*m_swFoot*r^2*r0*cos(theta)*(x_M^2 + y_M^2)^(1/2) - 16*L_thigh*k0_ss*m_M*m_swFoot*r*x_M*(x_M^2 + y_M^2)^(1/2) - 16*L_thigh*k0_ss*m_swLeg*m_swFoot*r*x_M*(x_M^2 + y_M^2)^(1/2) - 6*L0_ss*L_thigh^2*k0_ss*m_swLeg*m_swFoot*x_M*cos(theta)^2 - 3*L0_ss*L_thigh^2*k0_ss*m_swLeg*m_swFoot*y_M*sin(2*theta) + 4*L_thigh^3*dtheta^2*m_M*m_swLeg*m_swFoot*cos(theta)*(x_M^2 + y_M^2)^(1/2) - 4*L_thigh^2*dr*dtheta*m_swLeg^2*m_swFoot*sin(theta)*(x_M^2 + y_M^2)^(1/2) + 6*L_thigh^2*k0_ss*m_swLeg*m_swFoot*x_M*cos(theta)^2*(x_M^2 + y_M^2)^(1/2) + 3*L_thigh^2*k0_ss*m_swLeg*m_swFoot*y_M*sin(2*theta)*(x_M^2 + y_M^2)^(1/2) + 16*I_swLeg*dr*dtheta*m_M*m_swFoot*sin(theta)*(x_M^2 + y_M^2)^(1/2) + 16*I_swFoot*dr*dtheta*m_M*m_swFoot*sin(theta)*(x_M^2 + y_M^2)^(1/2) + 16*I_swLeg*dr*dtheta*m_swLeg*m_swFoot*sin(theta)*(x_M^2 + y_M^2)^(1/2) + 16*I_swFoot*dr*dtheta*m_swLeg*m_swFoot*sin(theta)*(x_M^2 + y_M^2)^(1/2) - 4*L_thigh*k_swLeg*m_M*m_swLeg*theta*sin(theta)*(x_M^2 + y_M^2)^(1/2) + 4*L_thigh*k_swLeg*m_M*m_swLeg*theta0*sin(theta)*(x_M^2 + y_M^2)^(1/2) - 8*L_thigh*k_swLeg*m_M*m_swFoot*theta*sin(theta)*(x_M^2 + y_M^2)^(1/2) + 8*L_thigh*k_swLeg*m_M*m_swFoot*theta0*sin(theta)*(x_M^2 + y_M^2)^(1/2) - 8*L_thigh*k_swLeg*m_swLeg*m_swFoot*theta*sin(theta)*(x_M^2 + y_M^2)^(1/2) + 8*L_thigh*k_swLeg*m_swLeg*m_swFoot*theta0*sin(theta)*(x_M^2 + y_M^2)^(1/2) + 4*L_thigh*dtheta^2*m_swLeg^2*m_swFoot*r^2*cos(theta)*(x_M^2 + y_M^2)^(1/2) + 4*L_thigh^2*dtheta^2*m_swLeg^2*m_swFoot*r*cos(theta)*(x_M^2 + y_M^2)^(1/2) + 4*I_swLeg*L_thigh*dtheta^2*m_M*m_swLeg*cos(theta)*(x_M^2 + y_M^2)^(1/2) + 4*I_swFoot*L_thigh*dtheta^2*m_M*m_swLeg*cos(theta)*(x_M^2 + y_M^2)^(1/2) + 4*I_swLeg*L_thigh*dtheta^2*m_swLeg*m_swFoot*cos(theta)*(x_M^2 + y_M^2)^(1/2) + 4*I_swFoot*L_thigh*dtheta^2*m_swLeg*m_swFoot*cos(theta)*(x_M^2 + y_M^2)^(1/2) - 8*k_swLeg*m_M*m_swFoot*r*theta*sin(theta)*(x_M^2 + y_M^2)^(1/2) + 8*k_swLeg*m_M*m_swFoot*r*theta0*sin(theta)*(x_M^2 + y_M^2)^(1/2) - 8*k_swLeg*m_swLeg*m_swFoot*r*theta*sin(theta)*(x_M^2 + y_M^2)^(1/2) + 8*k_swLeg*m_swLeg*m_swFoot*r*theta0*sin(theta)*(x_M^2 + y_M^2)^(1/2) - 16*L_thigh*k_swFoot*m_M*m_swFoot*r*r0*cos(theta)*(x_M^2 + y_M^2)^(1/2) - 8*L_thigh*k_swFoot*m_swLeg*m_swFoot*r*r0*cos(theta)*(x_M^2 + y_M^2)^(1/2) - 8*L0_ss*L_thigh*k0_ss*m_swLeg*m_swFoot*r*x_M*cos(theta)^2 - 4*L0_ss*L_thigh*k0_ss*m_swLeg*m_swFoot*r*y_M*sin(2*theta) - 4*L_thigh^2*dr*dtheta*m_M*m_swLeg*m_swFoot*sin(theta)*(x_M^2 + y_M^2)^(1/2) - 8*L_thigh*dr*dtheta*m_swLeg^2*m_swFoot*r*sin(theta)*(x_M^2 + y_M^2)^(1/2) + 8*L_thigh*k0_ss*m_swLeg*m_swFoot*r*x_M*cos(theta)^2*(x_M^2 + y_M^2)^(1/2) + 4*L_thigh*k0_ss*m_swLeg*m_swFoot*r*y_M*sin(2*theta)*(x_M^2 + y_M^2)^(1/2) + 4*L_thigh*dtheta^2*m_M*m_swLeg*m_swFoot*r^2*cos(theta)*(x_M^2 + y_M^2)^(1/2) + 8*L_thigh^2*dtheta^2*m_M*m_swLeg*m_swFoot*r*cos(theta)*(x_M^2 + y_M^2)^(1/2) - 8*L_thigh*dr*dtheta*m_M*m_swLeg*m_swFoot*r*sin(theta)*(x_M^2 + y_M^2)^(1/2)))/(2*(x_M^2 + y_M^2)^(1/2)*(m_M + m_swLeg)*(4*I_swLeg*m_M + 4*I_swFoot*m_M + 4*I_swLeg*m_swLeg + 4*I_swLeg*m_swFoot + 4*I_swFoot*m_swLeg + 4*I_swFoot*m_swFoot + 4*m_M*m_swFoot*r^2 + 4*m_swLeg*m_swFoot*r^2 + L_thigh^2*m_M*m_swLeg + 4*L_thigh^2*m_M*m_swFoot + L_thigh^2*m_swLeg*m_swFoot + 8*L_thigh*m_M*m_swFoot*r + 4*L_thigh*m_swLeg*m_swFoot*r));
            del2_x_swFoot_star*dx_M^2 + dtheta*(dr*sin(theta) + dtheta*cos(theta)*(L_thigh + r)) - K_p*(x_M - x_swFoot_star + cos(theta)*(L_thigh + r)) + K_d*(dx_M*(del_x_swFoot_star - 1) - dr*cos(theta) + dtheta*sin(theta)*(L_thigh + r)) + dr*dtheta*sin(theta) + ((del_x_swFoot_star - 1)*(2*L0_ss*L_thigh^2*k0_ss*m_swLeg^2*x_M - 2*L_thigh^2*k0_ss*m_swLeg^2*x_M*(x_M^2 + y_M^2)^(1/2) + 8*I_swLeg*L0_ss*k0_ss*m_M*x_M + 8*I_swFoot*L0_ss*k0_ss*m_M*x_M + 8*I_swLeg*L0_ss*k0_ss*m_swLeg*x_M + 8*I_swFoot*L0_ss*k0_ss*m_swLeg*x_M - 8*I_swLeg*k0_ss*m_M*x_M*(x_M^2 + y_M^2)^(1/2) - 8*I_swFoot*k0_ss*m_M*x_M*(x_M^2 + y_M^2)^(1/2) - 8*I_swLeg*k0_ss*m_swLeg*x_M*(x_M^2 + y_M^2)^(1/2) - 8*I_swFoot*k0_ss*m_swLeg*x_M*(x_M^2 + y_M^2)^(1/2) + 2*L0_ss*L_thigh^2*k0_ss*m_M*m_swLeg*x_M + 8*L0_ss*L_thigh^2*k0_ss*m_M*m_swFoot*x_M + 8*L0_ss*L_thigh^2*k0_ss*m_swLeg*m_swFoot*x_M - 2*L_thigh^2*k0_ss*m_M*m_swLeg*x_M*(x_M^2 + y_M^2)^(1/2) - 8*L_thigh^2*k0_ss*m_M*m_swFoot*x_M*(x_M^2 + y_M^2)^(1/2) - 8*L_thigh^2*k0_ss*m_swLeg*m_swFoot*x_M*(x_M^2 + y_M^2)^(1/2) + 8*I_swLeg*k_swFoot*m_M*r*cos(theta)*(x_M^2 + y_M^2)^(1/2) - 8*I_swLeg*k_swFoot*m_M*r0*cos(theta)*(x_M^2 + y_M^2)^(1/2) + 8*I_swFoot*k_swFoot*m_M*r*cos(theta)*(x_M^2 + y_M^2)^(1/2) - 8*I_swFoot*k_swFoot*m_M*r0*cos(theta)*(x_M^2 + y_M^2)^(1/2) + 8*I_swLeg*k_swFoot*m_swLeg*r*cos(theta)*(x_M^2 + y_M^2)^(1/2) - 8*I_swLeg*k_swFoot*m_swLeg*r0*cos(theta)*(x_M^2 + y_M^2)^(1/2) + 8*I_swLeg*k_swFoot*m_swFoot*r*cos(theta)*(x_M^2 + y_M^2)^(1/2) - 8*I_swLeg*k_swFoot*m_swFoot*r0*cos(theta)*(x_M^2 + y_M^2)^(1/2) + 8*I_swFoot*k_swFoot*m_swLeg*r*cos(theta)*(x_M^2 + y_M^2)^(1/2) - 8*I_swFoot*k_swFoot*m_swLeg*r0*cos(theta)*(x_M^2 + y_M^2)^(1/2) + 8*I_swFoot*k_swFoot*m_swFoot*r*cos(theta)*(x_M^2 + y_M^2)^(1/2) - 8*I_swFoot*k_swFoot*m_swFoot*r0*cos(theta)*(x_M^2 + y_M^2)^(1/2) + 8*L0_ss*k0_ss*m_M*m_swFoot*r^2*x_M + 8*L0_ss*k0_ss*m_swLeg*m_swFoot*r^2*x_M - 2*L0_ss*L_thigh^2*k0_ss*m_swLeg^2*x_M*cos(theta)^2 - L0_ss*L_thigh^2*k0_ss*m_swLeg^2*y_M*sin(2*theta) + L_thigh^3*dtheta^2*m_M*m_swLeg^2*cos(theta)*(x_M^2 + y_M^2)^(1/2) + L_thigh^3*dtheta^2*m_swLeg^2*m_swFoot*cos(theta)*(x_M^2 + y_M^2)^(1/2) - 8*k0_ss*m_M*m_swFoot*r^2*x_M*(x_M^2 + y_M^2)^(1/2) - 8*k0_ss*m_swLeg*m_swFoot*r^2*x_M*(x_M^2 + y_M^2)^(1/2) + 2*L_thigh^2*k0_ss*m_swLeg^2*x_M*cos(theta)^2*(x_M^2 + y_M^2)^(1/2) + L_thigh^2*k0_ss*m_swLeg^2*y_M*sin(2*theta)*(x_M^2 + y_M^2)^(1/2) + 8*I_swLeg*L0_ss*k0_ss*m_swFoot*x_M*cos(theta)^2 + 8*I_swFoot*L0_ss*k0_ss*m_swFoot*x_M*cos(theta)^2 + 4*I_swLeg*L0_ss*k0_ss*m_swFoot*y_M*sin(2*theta) + 4*I_swFoot*L0_ss*k0_ss*m_swFoot*y_M*sin(2*theta) - 8*I_swLeg*k0_ss*m_swFoot*x_M*cos(theta)^2*(x_M^2 + y_M^2)^(1/2) - 8*I_swFoot*k0_ss*m_swFoot*x_M*cos(theta)^2*(x_M^2 + y_M^2)^(1/2) - 4*L_thigh*k_swLeg*m_swLeg^2*theta*sin(theta)*(x_M^2 + y_M^2)^(1/2) + 4*L_thigh*k_swLeg*m_swLeg^2*theta0*sin(theta)*(x_M^2 + y_M^2)^(1/2) - 4*I_swLeg*k0_ss*m_swFoot*y_M*sin(2*theta)*(x_M^2 + y_M^2)^(1/2) - 4*I_swFoot*k0_ss*m_swFoot*y_M*sin(2*theta)*(x_M^2 + y_M^2)^(1/2) + 8*k_swFoot*m_M*m_swFoot*r^3*cos(theta)*(x_M^2 + y_M^2)^(1/2) + 8*k_swFoot*m_swLeg*m_swFoot*r^3*cos(theta)*(x_M^2 + y_M^2)^(1/2) + 4*I_swLeg*L_thigh*dtheta^2*m_swLeg^2*cos(theta)*(x_M^2 + y_M^2)^(1/2) + 4*I_swFoot*L_thigh*dtheta^2*m_swLeg^2*cos(theta)*(x_M^2 + y_M^2)^(1/2) + 2*L_thigh^2*k_swFoot*m_M*m_swLeg*r*cos(theta)*(x_M^2 + y_M^2)^(1/2) - 2*L_thigh^2*k_swFoot*m_M*m_swLeg*r0*cos(theta)*(x_M^2 + y_M^2)^(1/2) + 16*L_thigh*k_swFoot*m_M*m_swFoot*r^2*cos(theta)*(x_M^2 + y_M^2)^(1/2) + 8*L_thigh^2*k_swFoot*m_M*m_swFoot*r*cos(theta)*(x_M^2 + y_M^2)^(1/2) - 8*L_thigh^2*k_swFoot*m_M*m_swFoot*r0*cos(theta)*(x_M^2 + y_M^2)^(1/2) + 8*L_thigh*k_swFoot*m_swLeg*m_swFoot*r^2*cos(theta)*(x_M^2 + y_M^2)^(1/2) + 2*L_thigh^2*k_swFoot*m_swLeg*m_swFoot*r*cos(theta)*(x_M^2 + y_M^2)^(1/2) - 2*L_thigh^2*k_swFoot*m_swLeg*m_swFoot*r0*cos(theta)*(x_M^2 + y_M^2)^(1/2) + 16*L0_ss*L_thigh*k0_ss*m_M*m_swFoot*r*x_M + 16*L0_ss*L_thigh*k0_ss*m_swLeg*m_swFoot*r*x_M - 8*k_swFoot*m_M*m_swFoot*r^2*r0*cos(theta)*(x_M^2 + y_M^2)^(1/2) - 8*k_swFoot*m_swLeg*m_swFoot*r^2*r0*cos(theta)*(x_M^2 + y_M^2)^(1/2) - 16*L_thigh*k0_ss*m_M*m_swFoot*r*x_M*(x_M^2 + y_M^2)^(1/2) - 16*L_thigh*k0_ss*m_swLeg*m_swFoot*r*x_M*(x_M^2 + y_M^2)^(1/2) - 6*L0_ss*L_thigh^2*k0_ss*m_swLeg*m_swFoot*x_M*cos(theta)^2 - 3*L0_ss*L_thigh^2*k0_ss*m_swLeg*m_swFoot*y_M*sin(2*theta) + 4*L_thigh^3*dtheta^2*m_M*m_swLeg*m_swFoot*cos(theta)*(x_M^2 + y_M^2)^(1/2) - 4*L_thigh^2*dr*dtheta*m_swLeg^2*m_swFoot*sin(theta)*(x_M^2 + y_M^2)^(1/2) + 6*L_thigh^2*k0_ss*m_swLeg*m_swFoot*x_M*cos(theta)^2*(x_M^2 + y_M^2)^(1/2) + 3*L_thigh^2*k0_ss*m_swLeg*m_swFoot*y_M*sin(2*theta)*(x_M^2 + y_M^2)^(1/2) + 16*I_swLeg*dr*dtheta*m_M*m_swFoot*sin(theta)*(x_M^2 + y_M^2)^(1/2) + 16*I_swFoot*dr*dtheta*m_M*m_swFoot*sin(theta)*(x_M^2 + y_M^2)^(1/2) + 16*I_swLeg*dr*dtheta*m_swLeg*m_swFoot*sin(theta)*(x_M^2 + y_M^2)^(1/2) + 16*I_swFoot*dr*dtheta*m_swLeg*m_swFoot*sin(theta)*(x_M^2 + y_M^2)^(1/2) - 4*L_thigh*k_swLeg*m_M*m_swLeg*theta*sin(theta)*(x_M^2 + y_M^2)^(1/2) + 4*L_thigh*k_swLeg*m_M*m_swLeg*theta0*sin(theta)*(x_M^2 + y_M^2)^(1/2) - 8*L_thigh*k_swLeg*m_M*m_swFoot*theta*sin(theta)*(x_M^2 + y_M^2)^(1/2) + 8*L_thigh*k_swLeg*m_M*m_swFoot*theta0*sin(theta)*(x_M^2 + y_M^2)^(1/2) - 8*L_thigh*k_swLeg*m_swLeg*m_swFoot*theta*sin(theta)*(x_M^2 + y_M^2)^(1/2) + 8*L_thigh*k_swLeg*m_swLeg*m_swFoot*theta0*sin(theta)*(x_M^2 + y_M^2)^(1/2) + 4*L_thigh*dtheta^2*m_swLeg^2*m_swFoot*r^2*cos(theta)*(x_M^2 + y_M^2)^(1/2) + 4*L_thigh^2*dtheta^2*m_swLeg^2*m_swFoot*r*cos(theta)*(x_M^2 + y_M^2)^(1/2) + 4*I_swLeg*L_thigh*dtheta^2*m_M*m_swLeg*cos(theta)*(x_M^2 + y_M^2)^(1/2) + 4*I_swFoot*L_thigh*dtheta^2*m_M*m_swLeg*cos(theta)*(x_M^2 + y_M^2)^(1/2) + 4*I_swLeg*L_thigh*dtheta^2*m_swLeg*m_swFoot*cos(theta)*(x_M^2 + y_M^2)^(1/2) + 4*I_swFoot*L_thigh*dtheta^2*m_swLeg*m_swFoot*cos(theta)*(x_M^2 + y_M^2)^(1/2) - 8*k_swLeg*m_M*m_swFoot*r*theta*sin(theta)*(x_M^2 + y_M^2)^(1/2) + 8*k_swLeg*m_M*m_swFoot*r*theta0*sin(theta)*(x_M^2 + y_M^2)^(1/2) - 8*k_swLeg*m_swLeg*m_swFoot*r*theta*sin(theta)*(x_M^2 + y_M^2)^(1/2) + 8*k_swLeg*m_swLeg*m_swFoot*r*theta0*sin(theta)*(x_M^2 + y_M^2)^(1/2) - 16*L_thigh*k_swFoot*m_M*m_swFoot*r*r0*cos(theta)*(x_M^2 + y_M^2)^(1/2) - 8*L_thigh*k_swFoot*m_swLeg*m_swFoot*r*r0*cos(theta)*(x_M^2 + y_M^2)^(1/2) - 8*L0_ss*L_thigh*k0_ss*m_swLeg*m_swFoot*r*x_M*cos(theta)^2 - 4*L0_ss*L_thigh*k0_ss*m_swLeg*m_swFoot*r*y_M*sin(2*theta) - 4*L_thigh^2*dr*dtheta*m_M*m_swLeg*m_swFoot*sin(theta)*(x_M^2 + y_M^2)^(1/2) - 8*L_thigh*dr*dtheta*m_swLeg^2*m_swFoot*r*sin(theta)*(x_M^2 + y_M^2)^(1/2) + 8*L_thigh*k0_ss*m_swLeg*m_swFoot*r*x_M*cos(theta)^2*(x_M^2 + y_M^2)^(1/2) + 4*L_thigh*k0_ss*m_swLeg*m_swFoot*r*y_M*sin(2*theta)*(x_M^2 + y_M^2)^(1/2) + 4*L_thigh*dtheta^2*m_M*m_swLeg*m_swFoot*r^2*cos(theta)*(x_M^2 + y_M^2)^(1/2) + 8*L_thigh^2*dtheta^2*m_M*m_swLeg*m_swFoot*r*cos(theta)*(x_M^2 + y_M^2)^(1/2) - 8*L_thigh*dr*dtheta*m_M*m_swLeg*m_swFoot*r*sin(theta)*(x_M^2 + y_M^2)^(1/2)))/(2*(x_M^2 + y_M^2)^(1/2)*(m_M + m_swLeg)*(4*I_swLeg*m_M + 4*I_swFoot*m_M + 4*I_swLeg*m_swLeg + 4*I_swLeg*m_swFoot + 4*I_swFoot*m_swLeg + 4*I_swFoot*m_swFoot + 4*m_M*m_swFoot*r^2 + 4*m_swLeg*m_swFoot*r^2 + L_thigh^2*m_M*m_swLeg + 4*L_thigh^2*m_M*m_swFoot + L_thigh^2*m_swLeg*m_swFoot + 8*L_thigh*m_M*m_swFoot*r + 4*L_thigh*m_swLeg*m_swFoot*r)) - (sin(theta)*(L_thigh + r)*(4*k_swLeg*m_M*theta*(x_M^2 + y_M^2)^(1/2) - 4*k_swLeg*m_M*theta0*(x_M^2 + y_M^2)^(1/2) + 4*k_swLeg*m_swLeg*theta*(x_M^2 + y_M^2)^(1/2) - 4*k_swLeg*m_swLeg*theta0*(x_M^2 + y_M^2)^(1/2) + 4*k_swLeg*m_swFoot*theta*(x_M^2 + y_M^2)^(1/2) - 4*k_swLeg*m_swFoot*theta0*(x_M^2 + y_M^2)^(1/2) + 2*L0_ss*L_thigh*k0_ss*m_swLeg*y_M*cos(theta) + 4*L0_ss*L_thigh*k0_ss*m_swFoot*y_M*cos(theta) - 2*L0_ss*L_thigh*k0_ss*m_swLeg*x_M*sin(theta) - 4*L0_ss*L_thigh*k0_ss*m_swFoot*x_M*sin(theta) - 2*L_thigh*k0_ss*m_swLeg*y_M*cos(theta)*(x_M^2 + y_M^2)^(1/2) - 4*L_thigh*k0_ss*m_swFoot*y_M*cos(theta)*(x_M^2 + y_M^2)^(1/2) + 4*L0_ss*k0_ss*m_swFoot*r*y_M*cos(theta) + 2*L_thigh*k0_ss*m_swLeg*x_M*sin(theta)*(x_M^2 + y_M^2)^(1/2) + 4*L_thigh*k0_ss*m_swFoot*x_M*sin(theta)*(x_M^2 + y_M^2)^(1/2) - 4*L0_ss*k0_ss*m_swFoot*r*x_M*sin(theta) - 4*k0_ss*m_swFoot*r*y_M*cos(theta)*(x_M^2 + y_M^2)^(1/2) + 4*k0_ss*m_swFoot*r*x_M*sin(theta)*(x_M^2 + y_M^2)^(1/2) + 8*L_thigh*dr*dtheta*m_M*m_swFoot*(x_M^2 + y_M^2)^(1/2) + 4*L_thigh*dr*dtheta*m_swLeg*m_swFoot*(x_M^2 + y_M^2)^(1/2) + 8*dr*dtheta*m_M*m_swFoot*r*(x_M^2 + y_M^2)^(1/2) + 8*dr*dtheta*m_swLeg*m_swFoot*r*(x_M^2 + y_M^2)^(1/2)))/((x_M^2 + y_M^2)^(1/2)*(4*I_swLeg*m_M + 4*I_swFoot*m_M + 4*I_swLeg*m_swLeg + 4*I_swLeg*m_swFoot + 4*I_swFoot*m_swLeg + 4*I_swFoot*m_swFoot + 4*m_M*m_swFoot*r^2 + 4*m_swLeg*m_swFoot*r^2 + L_thigh^2*m_M*m_swLeg + 4*L_thigh^2*m_M*m_swFoot + L_thigh^2*m_swLeg*m_swFoot + 8*L_thigh*m_M*m_swFoot*r + 4*L_thigh*m_swLeg*m_swFoot*r)) - (cos(theta)*(2*k_swFoot*m_M*r0*(x_M^2 + y_M^2)^(1/2) - 2*k_swFoot*m_M*r*(x_M^2 + y_M^2)^(1/2) - 2*k_swFoot*m_swLeg*r*(x_M^2 + y_M^2)^(1/2) + 2*k_swFoot*m_swLeg*r0*(x_M^2 + y_M^2)^(1/2) - 2*k_swFoot*m_swFoot*r*(x_M^2 + y_M^2)^(1/2) + 2*k_swFoot*m_swFoot*r0*(x_M^2 + y_M^2)^(1/2) + 2*k0_ss*m_swFoot*y_M*sin(theta)*(x_M^2 + y_M^2)^(1/2) + 2*L_thigh*dtheta^2*m_M*m_swFoot*(x_M^2 + y_M^2)^(1/2) + L_thigh*dtheta^2*m_swLeg*m_swFoot*(x_M^2 + y_M^2)^(1/2) - 2*L0_ss*k0_ss*m_swFoot*x_M*cos(theta) + 2*dtheta^2*m_M*m_swFoot*r*(x_M^2 + y_M^2)^(1/2) + 2*dtheta^2*m_swLeg*m_swFoot*r*(x_M^2 + y_M^2)^(1/2) - 2*L0_ss*k0_ss*m_swFoot*y_M*sin(theta) + 2*k0_ss*m_swFoot*x_M*cos(theta)*(x_M^2 + y_M^2)^(1/2)))/(2*m_swFoot*(x_M^2 + y_M^2)^(1/2)*(m_M + m_swLeg));
            del2_y_swFoot_star*dx_M^2 - dtheta*(dr*cos(theta) - dtheta*sin(theta)*(L_thigh + r)) - K_p*(y_M - y_swFoot_star + sin(theta)*(L_thigh + r)) - K_d*(dy_M - del_y_swFoot_star*dx_M + dr*sin(theta) + dtheta*cos(theta)*(L_thigh + r)) - dr*dtheta*cos(theta) + (8*I_swLeg*gravi*m_M^2*(x_M^2 + y_M^2)^(1/2) + 8*I_swFoot*gravi*m_M^2*(x_M^2 + y_M^2)^(1/2) + 8*I_swLeg*gravi*m_swLeg^2*(x_M^2 + y_M^2)^(1/2) + 8*I_swFoot*gravi*m_swLeg^2*(x_M^2 + y_M^2)^(1/2) - L0_ss*L_thigh^2*k0_ss*m_swLeg^2*y_M + 2*L_thigh^2*gravi*m_M*m_swLeg^2*(x_M^2 + y_M^2)^(1/2) + 2*L_thigh^2*gravi*m_M^2*m_swLeg*(x_M^2 + y_M^2)^(1/2) + 8*L_thigh^2*gravi*m_M^2*m_swFoot*(x_M^2 + y_M^2)^(1/2) + 2*L_thigh^2*gravi*m_swLeg^2*m_swFoot*(x_M^2 + y_M^2)^(1/2) + L_thigh^2*k0_ss*m_swLeg^2*y_M*(x_M^2 + y_M^2)^(1/2) + 8*gravi*m_M^2*m_swFoot*r^2*(x_M^2 + y_M^2)^(1/2) + 8*gravi*m_swLeg^2*m_swFoot*r^2*(x_M^2 + y_M^2)^(1/2) - 8*I_swLeg*L0_ss*k0_ss*m_M*y_M - 8*I_swFoot*L0_ss*k0_ss*m_M*y_M - 8*I_swLeg*L0_ss*k0_ss*m_swLeg*y_M - 4*I_swLeg*L0_ss*k0_ss*m_swFoot*y_M - 8*I_swFoot*L0_ss*k0_ss*m_swLeg*y_M - 4*I_swFoot*L0_ss*k0_ss*m_swFoot*y_M + 16*I_swLeg*gravi*m_M*m_swLeg*(x_M^2 + y_M^2)^(1/2) + 8*I_swLeg*gravi*m_M*m_swFoot*(x_M^2 + y_M^2)^(1/2) + 16*I_swFoot*gravi*m_M*m_swLeg*(x_M^2 + y_M^2)^(1/2) + 8*I_swFoot*gravi*m_M*m_swFoot*(x_M^2 + y_M^2)^(1/2) + 8*I_swLeg*gravi*m_swLeg*m_swFoot*(x_M^2 + y_M^2)^(1/2) + 8*I_swFoot*gravi*m_swLeg*m_swFoot*(x_M^2 + y_M^2)^(1/2) + 8*I_swLeg*k0_ss*m_M*y_M*(x_M^2 + y_M^2)^(1/2) + 8*I_swFoot*k0_ss*m_M*y_M*(x_M^2 + y_M^2)^(1/2) + 8*I_swLeg*k0_ss*m_swLeg*y_M*(x_M^2 + y_M^2)^(1/2) + 4*I_swLeg*k0_ss*m_swFoot*y_M*(x_M^2 + y_M^2)^(1/2) + 8*I_swFoot*k0_ss*m_swLeg*y_M*(x_M^2 + y_M^2)^(1/2) + 4*I_swFoot*k0_ss*m_swFoot*y_M*(x_M^2 + y_M^2)^(1/2) - 2*L0_ss*L_thigh^2*k0_ss*m_M*m_swLeg*y_M - 8*L0_ss*L_thigh^2*k0_ss*m_M*m_swFoot*y_M - 5*L0_ss*L_thigh^2*k0_ss*m_swLeg*m_swFoot*y_M + 10*L_thigh^2*gravi*m_M*m_swLeg*m_swFoot*(x_M^2 + y_M^2)^(1/2) + 16*L_thigh*gravi*m_M^2*m_swFoot*r*(x_M^2 + y_M^2)^(1/2) + 8*L_thigh*gravi*m_swLeg^2*m_swFoot*r*(x_M^2 + y_M^2)^(1/2) + 2*L_thigh^2*k0_ss*m_M*m_swLeg*y_M*(x_M^2 + y_M^2)^(1/2) + 8*L_thigh^2*k0_ss*m_M*m_swFoot*y_M*(x_M^2 + y_M^2)^(1/2) + 5*L_thigh^2*k0_ss*m_swLeg*m_swFoot*y_M*(x_M^2 + y_M^2)^(1/2) - 8*L0_ss*k0_ss*m_M*m_swFoot*r^2*y_M - 8*L0_ss*k0_ss*m_swLeg*m_swFoot*r^2*y_M - L0_ss*L_thigh^2*k0_ss*m_swLeg^2*y_M*cos(2*theta) - 8*I_swLeg*k_swFoot*m_M*r*sin(theta)*(x_M^2 + y_M^2)^(1/2) + 8*I_swLeg*k_swFoot*m_M*r0*sin(theta)*(x_M^2 + y_M^2)^(1/2) - 8*I_swFoot*k_swFoot*m_M*r*sin(theta)*(x_M^2 + y_M^2)^(1/2) + 8*I_swFoot*k_swFoot*m_M*r0*sin(theta)*(x_M^2 + y_M^2)^(1/2) - 8*I_swLeg*k_swFoot*m_swLeg*r*sin(theta)*(x_M^2 + y_M^2)^(1/2) + 8*I_swLeg*k_swFoot*m_swLeg*r0*sin(theta)*(x_M^2 + y_M^2)^(1/2) - 8*I_swLeg*k_swFoot*m_swFoot*r*sin(theta)*(x_M^2 + y_M^2)^(1/2) + 8*I_swLeg*k_swFoot*m_swFoot*r0*sin(theta)*(x_M^2 + y_M^2)^(1/2) - 8*I_swFoot*k_swFoot*m_swLeg*r*sin(theta)*(x_M^2 + y_M^2)^(1/2) + 8*I_swFoot*k_swFoot*m_swLeg*r0*sin(theta)*(x_M^2 + y_M^2)^(1/2) - 8*I_swFoot*k_swFoot*m_swFoot*r*sin(theta)*(x_M^2 + y_M^2)^(1/2) + 8*I_swFoot*k_swFoot*m_swFoot*r0*sin(theta)*(x_M^2 + y_M^2)^(1/2) + L0_ss*L_thigh^2*k0_ss*m_swLeg^2*x_M*sin(2*theta) + 16*gravi*m_M*m_swLeg*m_swFoot*r^2*(x_M^2 + y_M^2)^(1/2) + 8*k0_ss*m_M*m_swFoot*r^2*y_M*(x_M^2 + y_M^2)^(1/2) + 8*k0_ss*m_swLeg*m_swFoot*r^2*y_M*(x_M^2 + y_M^2)^(1/2) - L_thigh^3*dtheta^2*m_M*m_swLeg^2*sin(theta)*(x_M^2 + y_M^2)^(1/2) - L_thigh^3*dtheta^2*m_swLeg^2*m_swFoot*sin(theta)*(x_M^2 + y_M^2)^(1/2) + L_thigh^2*k0_ss*m_swLeg^2*y_M*cos(2*theta)*(x_M^2 + y_M^2)^(1/2) - L_thigh^2*k0_ss*m_swLeg^2*x_M*sin(2*theta)*(x_M^2 + y_M^2)^(1/2) + 4*I_swLeg*L0_ss*k0_ss*m_swFoot*y_M*cos(2*theta) + 4*I_swFoot*L0_ss*k0_ss*m_swFoot*y_M*cos(2*theta) - 4*I_swLeg*L0_ss*k0_ss*m_swFoot*x_M*sin(2*theta) - 4*I_swFoot*L0_ss*k0_ss*m_swFoot*x_M*sin(2*theta) - 4*L_thigh*k_swLeg*m_swLeg^2*theta*cos(theta)*(x_M^2 + y_M^2)^(1/2) + 4*L_thigh*k_swLeg*m_swLeg^2*theta0*cos(theta)*(x_M^2 + y_M^2)^(1/2) - 4*I_swLeg*k0_ss*m_swFoot*y_M*cos(2*theta)*(x_M^2 + y_M^2)^(1/2) - 4*I_swFoot*k0_ss*m_swFoot*y_M*cos(2*theta)*(x_M^2 + y_M^2)^(1/2) + 4*I_swLeg*k0_ss*m_swFoot*x_M*sin(2*theta)*(x_M^2 + y_M^2)^(1/2) + 4*I_swFoot*k0_ss*m_swFoot*x_M*sin(2*theta)*(x_M^2 + y_M^2)^(1/2) - 8*k_swFoot*m_M*m_swFoot*r^3*sin(theta)*(x_M^2 + y_M^2)^(1/2) - 8*k_swFoot*m_swLeg*m_swFoot*r^3*sin(theta)*(x_M^2 + y_M^2)^(1/2) - 4*I_swLeg*L_thigh*dtheta^2*m_swLeg^2*sin(theta)*(x_M^2 + y_M^2)^(1/2) - 4*I_swFoot*L_thigh*dtheta^2*m_swLeg^2*sin(theta)*(x_M^2 + y_M^2)^(1/2) - 2*L_thigh^2*k_swFoot*m_M*m_swLeg*r*sin(theta)*(x_M^2 + y_M^2)^(1/2) + 2*L_thigh^2*k_swFoot*m_M*m_swLeg*r0*sin(theta)*(x_M^2 + y_M^2)^(1/2) - 16*L_thigh*k_swFoot*m_M*m_swFoot*r^2*sin(theta)*(x_M^2 + y_M^2)^(1/2) - 8*L_thigh^2*k_swFoot*m_M*m_swFoot*r*sin(theta)*(x_M^2 + y_M^2)^(1/2) + 8*L_thigh^2*k_swFoot*m_M*m_swFoot*r0*sin(theta)*(x_M^2 + y_M^2)^(1/2) - 8*L_thigh*k_swFoot*m_swLeg*m_swFoot*r^2*sin(theta)*(x_M^2 + y_M^2)^(1/2) - 2*L_thigh^2*k_swFoot*m_swLeg*m_swFoot*r*sin(theta)*(x_M^2 + y_M^2)^(1/2) + 2*L_thigh^2*k_swFoot*m_swLeg*m_swFoot*r0*sin(theta)*(x_M^2 + y_M^2)^(1/2) - 16*L0_ss*L_thigh*k0_ss*m_M*m_swFoot*r*y_M - 12*L0_ss*L_thigh*k0_ss*m_swLeg*m_swFoot*r*y_M + 24*L_thigh*gravi*m_M*m_swLeg*m_swFoot*r*(x_M^2 + y_M^2)^(1/2) + 8*k_swFoot*m_M*m_swFoot*r^2*r0*sin(theta)*(x_M^2 + y_M^2)^(1/2) + 8*k_swFoot*m_swLeg*m_swFoot*r^2*r0*sin(theta)*(x_M^2 + y_M^2)^(1/2) + 16*L_thigh*k0_ss*m_M*m_swFoot*r*y_M*(x_M^2 + y_M^2)^(1/2) + 12*L_thigh*k0_ss*m_swLeg*m_swFoot*r*y_M*(x_M^2 + y_M^2)^(1/2) - 3*L0_ss*L_thigh^2*k0_ss*m_swLeg*m_swFoot*y_M*cos(2*theta) - 4*L_thigh^2*dr*dtheta*m_swLeg^2*m_swFoot*cos(theta)*(x_M^2 + y_M^2)^(1/2) + 3*L0_ss*L_thigh^2*k0_ss*m_swLeg*m_swFoot*x_M*sin(2*theta) - 4*L_thigh^3*dtheta^2*m_M*m_swLeg*m_swFoot*sin(theta)*(x_M^2 + y_M^2)^(1/2) + 3*L_thigh^2*k0_ss*m_swLeg*m_swFoot*y_M*cos(2*theta)*(x_M^2 + y_M^2)^(1/2) - 3*L_thigh^2*k0_ss*m_swLeg*m_swFoot*x_M*sin(2*theta)*(x_M^2 + y_M^2)^(1/2) + 16*I_swLeg*dr*dtheta*m_M*m_swFoot*cos(theta)*(x_M^2 + y_M^2)^(1/2) + 16*I_swFoot*dr*dtheta*m_M*m_swFoot*cos(theta)*(x_M^2 + y_M^2)^(1/2) + 16*I_swLeg*dr*dtheta*m_swLeg*m_swFoot*cos(theta)*(x_M^2 + y_M^2)^(1/2) + 16*I_swFoot*dr*dtheta*m_swLeg*m_swFoot*cos(theta)*(x_M^2 + y_M^2)^(1/2) - 4*L_thigh*k_swLeg*m_M*m_swLeg*theta*cos(theta)*(x_M^2 + y_M^2)^(1/2) + 4*L_thigh*k_swLeg*m_M*m_swLeg*theta0*cos(theta)*(x_M^2 + y_M^2)^(1/2) - 8*L_thigh*k_swLeg*m_M*m_swFoot*theta*cos(theta)*(x_M^2 + y_M^2)^(1/2) + 8*L_thigh*k_swLeg*m_M*m_swFoot*theta0*cos(theta)*(x_M^2 + y_M^2)^(1/2) - 8*L_thigh*k_swLeg*m_swLeg*m_swFoot*theta*cos(theta)*(x_M^2 + y_M^2)^(1/2) + 8*L_thigh*k_swLeg*m_swLeg*m_swFoot*theta0*cos(theta)*(x_M^2 + y_M^2)^(1/2) - 4*L_thigh*dtheta^2*m_swLeg^2*m_swFoot*r^2*sin(theta)*(x_M^2 + y_M^2)^(1/2) - 4*L_thigh^2*dtheta^2*m_swLeg^2*m_swFoot*r*sin(theta)*(x_M^2 + y_M^2)^(1/2) - 8*k_swLeg*m_M*m_swFoot*r*theta*cos(theta)*(x_M^2 + y_M^2)^(1/2) + 8*k_swLeg*m_M*m_swFoot*r*theta0*cos(theta)*(x_M^2 + y_M^2)^(1/2) - 8*k_swLeg*m_swLeg*m_swFoot*r*theta*cos(theta)*(x_M^2 + y_M^2)^(1/2) + 8*k_swLeg*m_swLeg*m_swFoot*r*theta0*cos(theta)*(x_M^2 + y_M^2)^(1/2) - 4*I_swLeg*L_thigh*dtheta^2*m_M*m_swLeg*sin(theta)*(x_M^2 + y_M^2)^(1/2) - 4*I_swFoot*L_thigh*dtheta^2*m_M*m_swLeg*sin(theta)*(x_M^2 + y_M^2)^(1/2) - 4*I_swLeg*L_thigh*dtheta^2*m_swLeg*m_swFoot*sin(theta)*(x_M^2 + y_M^2)^(1/2) - 4*I_swFoot*L_thigh*dtheta^2*m_swLeg*m_swFoot*sin(theta)*(x_M^2 + y_M^2)^(1/2) + 16*L_thigh*k_swFoot*m_M*m_swFoot*r*r0*sin(theta)*(x_M^2 + y_M^2)^(1/2) + 8*L_thigh*k_swFoot*m_swLeg*m_swFoot*r*r0*sin(theta)*(x_M^2 + y_M^2)^(1/2) - 4*L0_ss*L_thigh*k0_ss*m_swLeg*m_swFoot*r*y_M*cos(2*theta) - 4*L_thigh^2*dr*dtheta*m_M*m_swLeg*m_swFoot*cos(theta)*(x_M^2 + y_M^2)^(1/2) - 8*L_thigh*dr*dtheta*m_swLeg^2*m_swFoot*r*cos(theta)*(x_M^2 + y_M^2)^(1/2) + 4*L0_ss*L_thigh*k0_ss*m_swLeg*m_swFoot*r*x_M*sin(2*theta) + 4*L_thigh*k0_ss*m_swLeg*m_swFoot*r*y_M*cos(2*theta)*(x_M^2 + y_M^2)^(1/2) - 4*L_thigh*k0_ss*m_swLeg*m_swFoot*r*x_M*sin(2*theta)*(x_M^2 + y_M^2)^(1/2) - 4*L_thigh*dtheta^2*m_M*m_swLeg*m_swFoot*r^2*sin(theta)*(x_M^2 + y_M^2)^(1/2) - 8*L_thigh^2*dtheta^2*m_M*m_swLeg*m_swFoot*r*sin(theta)*(x_M^2 + y_M^2)^(1/2) - 8*L_thigh*dr*dtheta*m_M*m_swLeg*m_swFoot*r*cos(theta)*(x_M^2 + y_M^2)^(1/2))/(2*(x_M^2 + y_M^2)^(1/2)*(m_M + m_swLeg)*(4*I_swLeg*m_M + 4*I_swFoot*m_M + 4*I_swLeg*m_swLeg + 4*I_swLeg*m_swFoot + 4*I_swFoot*m_swLeg + 4*I_swFoot*m_swFoot + 4*m_M*m_swFoot*r^2 + 4*m_swLeg*m_swFoot*r^2 + L_thigh^2*m_M*m_swLeg + 4*L_thigh^2*m_M*m_swFoot + L_thigh^2*m_swLeg*m_swFoot + 8*L_thigh*m_M*m_swFoot*r + 4*L_thigh*m_swLeg*m_swFoot*r)) - (sin(theta)*(2*k_swFoot*m_M*r0*(x_M^2 + y_M^2)^(1/2) - 2*k_swFoot*m_M*r*(x_M^2 + y_M^2)^(1/2) - 2*k_swFoot*m_swLeg*r*(x_M^2 + y_M^2)^(1/2) + 2*k_swFoot*m_swLeg*r0*(x_M^2 + y_M^2)^(1/2) - 2*k_swFoot*m_swFoot*r*(x_M^2 + y_M^2)^(1/2) + 2*k_swFoot*m_swFoot*r0*(x_M^2 + y_M^2)^(1/2) + 2*k0_ss*m_swFoot*y_M*sin(theta)*(x_M^2 + y_M^2)^(1/2) + 2*L_thigh*dtheta^2*m_M*m_swFoot*(x_M^2 + y_M^2)^(1/2) + L_thigh*dtheta^2*m_swLeg*m_swFoot*(x_M^2 + y_M^2)^(1/2) - 2*L0_ss*k0_ss*m_swFoot*x_M*cos(theta) + 2*dtheta^2*m_M*m_swFoot*r*(x_M^2 + y_M^2)^(1/2) + 2*dtheta^2*m_swLeg*m_swFoot*r*(x_M^2 + y_M^2)^(1/2) - 2*L0_ss*k0_ss*m_swFoot*y_M*sin(theta) + 2*k0_ss*m_swFoot*x_M*cos(theta)*(x_M^2 + y_M^2)^(1/2)))/(2*m_swFoot*(x_M^2 + y_M^2)^(1/2)*(m_M + m_swLeg)) + (cos(theta)*(L_thigh + r)*(4*k_swLeg*m_M*theta*(x_M^2 + y_M^2)^(1/2) - 4*k_swLeg*m_M*theta0*(x_M^2 + y_M^2)^(1/2) + 4*k_swLeg*m_swLeg*theta*(x_M^2 + y_M^2)^(1/2) - 4*k_swLeg*m_swLeg*theta0*(x_M^2 + y_M^2)^(1/2) + 4*k_swLeg*m_swFoot*theta*(x_M^2 + y_M^2)^(1/2) - 4*k_swLeg*m_swFoot*theta0*(x_M^2 + y_M^2)^(1/2) + 2*L0_ss*L_thigh*k0_ss*m_swLeg*y_M*cos(theta) + 4*L0_ss*L_thigh*k0_ss*m_swFoot*y_M*cos(theta) - 2*L0_ss*L_thigh*k0_ss*m_swLeg*x_M*sin(theta) - 4*L0_ss*L_thigh*k0_ss*m_swFoot*x_M*sin(theta) - 2*L_thigh*k0_ss*m_swLeg*y_M*cos(theta)*(x_M^2 + y_M^2)^(1/2) - 4*L_thigh*k0_ss*m_swFoot*y_M*cos(theta)*(x_M^2 + y_M^2)^(1/2) + 4*L0_ss*k0_ss*m_swFoot*r*y_M*cos(theta) + 2*L_thigh*k0_ss*m_swLeg*x_M*sin(theta)*(x_M^2 + y_M^2)^(1/2) + 4*L_thigh*k0_ss*m_swFoot*x_M*sin(theta)*(x_M^2 + y_M^2)^(1/2) - 4*L0_ss*k0_ss*m_swFoot*r*x_M*sin(theta) - 4*k0_ss*m_swFoot*r*y_M*cos(theta)*(x_M^2 + y_M^2)^(1/2) + 4*k0_ss*m_swFoot*r*x_M*sin(theta)*(x_M^2 + y_M^2)^(1/2) + 8*L_thigh*dr*dtheta*m_M*m_swFoot*(x_M^2 + y_M^2)^(1/2) + 4*L_thigh*dr*dtheta*m_swLeg*m_swFoot*(x_M^2 + y_M^2)^(1/2) + 8*dr*dtheta*m_M*m_swFoot*r*(x_M^2 + y_M^2)^(1/2) + 8*dr*dtheta*m_swLeg*m_swFoot*r*(x_M^2 + y_M^2)^(1/2)))/((x_M^2 + y_M^2)^(1/2)*(4*I_swLeg*m_M + 4*I_swFoot*m_M + 4*I_swLeg*m_swLeg + 4*I_swLeg*m_swFoot + 4*I_swFoot*m_swLeg + 4*I_swFoot*m_swFoot + 4*m_M*m_swFoot*r^2 + 4*m_swLeg*m_swFoot*r^2 + L_thigh^2*m_M*m_swLeg + 4*L_thigh^2*m_M*m_swFoot + L_thigh^2*m_swLeg*m_swFoot + 8*L_thigh*m_M*m_swFoot*r + 4*L_thigh*m_swLeg*m_swFoot*r)) + (del_y_swFoot_star*(2*L0_ss*L_thigh^2*k0_ss*m_swLeg^2*x_M - 2*L_thigh^2*k0_ss*m_swLeg^2*x_M*(x_M^2 + y_M^2)^(1/2) + 8*I_swLeg*L0_ss*k0_ss*m_M*x_M + 8*I_swFoot*L0_ss*k0_ss*m_M*x_M + 8*I_swLeg*L0_ss*k0_ss*m_swLeg*x_M + 8*I_swFoot*L0_ss*k0_ss*m_swLeg*x_M - 8*I_swLeg*k0_ss*m_M*x_M*(x_M^2 + y_M^2)^(1/2) - 8*I_swFoot*k0_ss*m_M*x_M*(x_M^2 + y_M^2)^(1/2) - 8*I_swLeg*k0_ss*m_swLeg*x_M*(x_M^2 + y_M^2)^(1/2) - 8*I_swFoot*k0_ss*m_swLeg*x_M*(x_M^2 + y_M^2)^(1/2) + 2*L0_ss*L_thigh^2*k0_ss*m_M*m_swLeg*x_M + 8*L0_ss*L_thigh^2*k0_ss*m_M*m_swFoot*x_M + 8*L0_ss*L_thigh^2*k0_ss*m_swLeg*m_swFoot*x_M - 2*L_thigh^2*k0_ss*m_M*m_swLeg*x_M*(x_M^2 + y_M^2)^(1/2) - 8*L_thigh^2*k0_ss*m_M*m_swFoot*x_M*(x_M^2 + y_M^2)^(1/2) - 8*L_thigh^2*k0_ss*m_swLeg*m_swFoot*x_M*(x_M^2 + y_M^2)^(1/2) + 8*I_swLeg*k_swFoot*m_M*r*cos(theta)*(x_M^2 + y_M^2)^(1/2) - 8*I_swLeg*k_swFoot*m_M*r0*cos(theta)*(x_M^2 + y_M^2)^(1/2) + 8*I_swFoot*k_swFoot*m_M*r*cos(theta)*(x_M^2 + y_M^2)^(1/2) - 8*I_swFoot*k_swFoot*m_M*r0*cos(theta)*(x_M^2 + y_M^2)^(1/2) + 8*I_swLeg*k_swFoot*m_swLeg*r*cos(theta)*(x_M^2 + y_M^2)^(1/2) - 8*I_swLeg*k_swFoot*m_swLeg*r0*cos(theta)*(x_M^2 + y_M^2)^(1/2) + 8*I_swLeg*k_swFoot*m_swFoot*r*cos(theta)*(x_M^2 + y_M^2)^(1/2) - 8*I_swLeg*k_swFoot*m_swFoot*r0*cos(theta)*(x_M^2 + y_M^2)^(1/2) + 8*I_swFoot*k_swFoot*m_swLeg*r*cos(theta)*(x_M^2 + y_M^2)^(1/2) - 8*I_swFoot*k_swFoot*m_swLeg*r0*cos(theta)*(x_M^2 + y_M^2)^(1/2) + 8*I_swFoot*k_swFoot*m_swFoot*r*cos(theta)*(x_M^2 + y_M^2)^(1/2) - 8*I_swFoot*k_swFoot*m_swFoot*r0*cos(theta)*(x_M^2 + y_M^2)^(1/2) + 8*L0_ss*k0_ss*m_M*m_swFoot*r^2*x_M + 8*L0_ss*k0_ss*m_swLeg*m_swFoot*r^2*x_M - 2*L0_ss*L_thigh^2*k0_ss*m_swLeg^2*x_M*cos(theta)^2 - L0_ss*L_thigh^2*k0_ss*m_swLeg^2*y_M*sin(2*theta) + L_thigh^3*dtheta^2*m_M*m_swLeg^2*cos(theta)*(x_M^2 + y_M^2)^(1/2) + L_thigh^3*dtheta^2*m_swLeg^2*m_swFoot*cos(theta)*(x_M^2 + y_M^2)^(1/2) - 8*k0_ss*m_M*m_swFoot*r^2*x_M*(x_M^2 + y_M^2)^(1/2) - 8*k0_ss*m_swLeg*m_swFoot*r^2*x_M*(x_M^2 + y_M^2)^(1/2) + 2*L_thigh^2*k0_ss*m_swLeg^2*x_M*cos(theta)^2*(x_M^2 + y_M^2)^(1/2) + L_thigh^2*k0_ss*m_swLeg^2*y_M*sin(2*theta)*(x_M^2 + y_M^2)^(1/2) + 8*I_swLeg*L0_ss*k0_ss*m_swFoot*x_M*cos(theta)^2 + 8*I_swFoot*L0_ss*k0_ss*m_swFoot*x_M*cos(theta)^2 + 4*I_swLeg*L0_ss*k0_ss*m_swFoot*y_M*sin(2*theta) + 4*I_swFoot*L0_ss*k0_ss*m_swFoot*y_M*sin(2*theta) - 8*I_swLeg*k0_ss*m_swFoot*x_M*cos(theta)^2*(x_M^2 + y_M^2)^(1/2) - 8*I_swFoot*k0_ss*m_swFoot*x_M*cos(theta)^2*(x_M^2 + y_M^2)^(1/2) - 4*L_thigh*k_swLeg*m_swLeg^2*theta*sin(theta)*(x_M^2 + y_M^2)^(1/2) + 4*L_thigh*k_swLeg*m_swLeg^2*theta0*sin(theta)*(x_M^2 + y_M^2)^(1/2) - 4*I_swLeg*k0_ss*m_swFoot*y_M*sin(2*theta)*(x_M^2 + y_M^2)^(1/2) - 4*I_swFoot*k0_ss*m_swFoot*y_M*sin(2*theta)*(x_M^2 + y_M^2)^(1/2) + 8*k_swFoot*m_M*m_swFoot*r^3*cos(theta)*(x_M^2 + y_M^2)^(1/2) + 8*k_swFoot*m_swLeg*m_swFoot*r^3*cos(theta)*(x_M^2 + y_M^2)^(1/2) + 4*I_swLeg*L_thigh*dtheta^2*m_swLeg^2*cos(theta)*(x_M^2 + y_M^2)^(1/2) + 4*I_swFoot*L_thigh*dtheta^2*m_swLeg^2*cos(theta)*(x_M^2 + y_M^2)^(1/2) + 2*L_thigh^2*k_swFoot*m_M*m_swLeg*r*cos(theta)*(x_M^2 + y_M^2)^(1/2) - 2*L_thigh^2*k_swFoot*m_M*m_swLeg*r0*cos(theta)*(x_M^2 + y_M^2)^(1/2) + 16*L_thigh*k_swFoot*m_M*m_swFoot*r^2*cos(theta)*(x_M^2 + y_M^2)^(1/2) + 8*L_thigh^2*k_swFoot*m_M*m_swFoot*r*cos(theta)*(x_M^2 + y_M^2)^(1/2) - 8*L_thigh^2*k_swFoot*m_M*m_swFoot*r0*cos(theta)*(x_M^2 + y_M^2)^(1/2) + 8*L_thigh*k_swFoot*m_swLeg*m_swFoot*r^2*cos(theta)*(x_M^2 + y_M^2)^(1/2) + 2*L_thigh^2*k_swFoot*m_swLeg*m_swFoot*r*cos(theta)*(x_M^2 + y_M^2)^(1/2) - 2*L_thigh^2*k_swFoot*m_swLeg*m_swFoot*r0*cos(theta)*(x_M^2 + y_M^2)^(1/2) + 16*L0_ss*L_thigh*k0_ss*m_M*m_swFoot*r*x_M + 16*L0_ss*L_thigh*k0_ss*m_swLeg*m_swFoot*r*x_M - 8*k_swFoot*m_M*m_swFoot*r^2*r0*cos(theta)*(x_M^2 + y_M^2)^(1/2) - 8*k_swFoot*m_swLeg*m_swFoot*r^2*r0*cos(theta)*(x_M^2 + y_M^2)^(1/2) - 16*L_thigh*k0_ss*m_M*m_swFoot*r*x_M*(x_M^2 + y_M^2)^(1/2) - 16*L_thigh*k0_ss*m_swLeg*m_swFoot*r*x_M*(x_M^2 + y_M^2)^(1/2) - 6*L0_ss*L_thigh^2*k0_ss*m_swLeg*m_swFoot*x_M*cos(theta)^2 - 3*L0_ss*L_thigh^2*k0_ss*m_swLeg*m_swFoot*y_M*sin(2*theta) + 4*L_thigh^3*dtheta^2*m_M*m_swLeg*m_swFoot*cos(theta)*(x_M^2 + y_M^2)^(1/2) - 4*L_thigh^2*dr*dtheta*m_swLeg^2*m_swFoot*sin(theta)*(x_M^2 + y_M^2)^(1/2) + 6*L_thigh^2*k0_ss*m_swLeg*m_swFoot*x_M*cos(theta)^2*(x_M^2 + y_M^2)^(1/2) + 3*L_thigh^2*k0_ss*m_swLeg*m_swFoot*y_M*sin(2*theta)*(x_M^2 + y_M^2)^(1/2) + 16*I_swLeg*dr*dtheta*m_M*m_swFoot*sin(theta)*(x_M^2 + y_M^2)^(1/2) + 16*I_swFoot*dr*dtheta*m_M*m_swFoot*sin(theta)*(x_M^2 + y_M^2)^(1/2) + 16*I_swLeg*dr*dtheta*m_swLeg*m_swFoot*sin(theta)*(x_M^2 + y_M^2)^(1/2) + 16*I_swFoot*dr*dtheta*m_swLeg*m_swFoot*sin(theta)*(x_M^2 + y_M^2)^(1/2) - 4*L_thigh*k_swLeg*m_M*m_swLeg*theta*sin(theta)*(x_M^2 + y_M^2)^(1/2) + 4*L_thigh*k_swLeg*m_M*m_swLeg*theta0*sin(theta)*(x_M^2 + y_M^2)^(1/2) - 8*L_thigh*k_swLeg*m_M*m_swFoot*theta*sin(theta)*(x_M^2 + y_M^2)^(1/2) + 8*L_thigh*k_swLeg*m_M*m_swFoot*theta0*sin(theta)*(x_M^2 + y_M^2)^(1/2) - 8*L_thigh*k_swLeg*m_swLeg*m_swFoot*theta*sin(theta)*(x_M^2 + y_M^2)^(1/2) + 8*L_thigh*k_swLeg*m_swLeg*m_swFoot*theta0*sin(theta)*(x_M^2 + y_M^2)^(1/2) + 4*L_thigh*dtheta^2*m_swLeg^2*m_swFoot*r^2*cos(theta)*(x_M^2 + y_M^2)^(1/2) + 4*L_thigh^2*dtheta^2*m_swLeg^2*m_swFoot*r*cos(theta)*(x_M^2 + y_M^2)^(1/2) + 4*I_swLeg*L_thigh*dtheta^2*m_M*m_swLeg*cos(theta)*(x_M^2 + y_M^2)^(1/2) + 4*I_swFoot*L_thigh*dtheta^2*m_M*m_swLeg*cos(theta)*(x_M^2 + y_M^2)^(1/2) + 4*I_swLeg*L_thigh*dtheta^2*m_swLeg*m_swFoot*cos(theta)*(x_M^2 + y_M^2)^(1/2) + 4*I_swFoot*L_thigh*dtheta^2*m_swLeg*m_swFoot*cos(theta)*(x_M^2 + y_M^2)^(1/2) - 8*k_swLeg*m_M*m_swFoot*r*theta*sin(theta)*(x_M^2 + y_M^2)^(1/2) + 8*k_swLeg*m_M*m_swFoot*r*theta0*sin(theta)*(x_M^2 + y_M^2)^(1/2) - 8*k_swLeg*m_swLeg*m_swFoot*r*theta*sin(theta)*(x_M^2 + y_M^2)^(1/2) + 8*k_swLeg*m_swLeg*m_swFoot*r*theta0*sin(theta)*(x_M^2 + y_M^2)^(1/2) - 16*L_thigh*k_swFoot*m_M*m_swFoot*r*r0*cos(theta)*(x_M^2 + y_M^2)^(1/2) - 8*L_thigh*k_swFoot*m_swLeg*m_swFoot*r*r0*cos(theta)*(x_M^2 + y_M^2)^(1/2) - 8*L0_ss*L_thigh*k0_ss*m_swLeg*m_swFoot*r*x_M*cos(theta)^2 - 4*L0_ss*L_thigh*k0_ss*m_swLeg*m_swFoot*r*y_M*sin(2*theta) - 4*L_thigh^2*dr*dtheta*m_M*m_swLeg*m_swFoot*sin(theta)*(x_M^2 + y_M^2)^(1/2) - 8*L_thigh*dr*dtheta*m_swLeg^2*m_swFoot*r*sin(theta)*(x_M^2 + y_M^2)^(1/2) + 8*L_thigh*k0_ss*m_swLeg*m_swFoot*r*x_M*cos(theta)^2*(x_M^2 + y_M^2)^(1/2) + 4*L_thigh*k0_ss*m_swLeg*m_swFoot*r*y_M*sin(2*theta)*(x_M^2 + y_M^2)^(1/2) + 4*L_thigh*dtheta^2*m_M*m_swLeg*m_swFoot*r^2*cos(theta)*(x_M^2 + y_M^2)^(1/2) + 8*L_thigh^2*dtheta^2*m_M*m_swLeg*m_swFoot*r*cos(theta)*(x_M^2 + y_M^2)^(1/2) - 8*L_thigh*dr*dtheta*m_M*m_swLeg*m_swFoot*r*sin(theta)*(x_M^2 + y_M^2)^(1/2)))/(2*(x_M^2 + y_M^2)^(1/2)*(m_M + m_swLeg)*(4*I_swLeg*m_M + 4*I_swFoot*m_M + 4*I_swLeg*m_swLeg + 4*I_swLeg*m_swFoot + 4*I_swFoot*m_swLeg + 4*I_swFoot*m_swFoot + 4*m_M*m_swFoot*r^2 + 4*m_swLeg*m_swFoot*r^2 + L_thigh^2*m_M*m_swLeg + 4*L_thigh^2*m_M*m_swFoot + L_thigh^2*m_swLeg*m_swFoot + 8*L_thigh*m_M*m_swFoot*r + 4*L_thigh*m_swLeg*m_swFoot*r))];

            % Regularitazation terms
            eps_ss = 1e-7;
            eps_1 = eps_ss/abs(det(A_ss));
            eps_2 = eps_ss/abs(det(A_ss));
            eps_3 = eps_ss/abs(det(A_ss));

            E_ss = [
            1/(eps_1 + 1),             0,             0;
            0, 1/(eps_2 + 1),             0;
            0,             0, 1/(eps_3 + 1)];

            % U_ss = (A_ss^-1)*K_ss;
            U_ss = E_ss*(A_ss^-1)*K_ss;

            det_A_ss = det(A_ss);

            u1 = U_ss(1);
            u2 = U_ss(2);
            u3 = U_ss(3);

            else
        ref_output_ss = [-1; -1; -1];
    end
else
    % if the system is in double stance phace

    if x_CoM_star_ds(1) <= x_CoM && x_CoM <= x_CoM_star_ds(end)

        % interpolation
        y_CoM_star = interp1(x_CoM_star_ds, ref_star_ds(:,2), x_CoM);
        dx_CoM_star = interp1(x_CoM_star_ds, ref_star_ds(:,3), x_CoM);

        del_y_CoM_star = interp1(x_CoM_star_ds, ref_star_ds(:,4), x_CoM);
        del_dx_CoM_star = interp1(x_CoM_star_ds, ref_star_ds(:,5), x_CoM);

        del2_y_CoM_star = interp1(x_CoM_star_ds, ref_star_ds(:,6), x_CoM);

        ref_output_ds = [y_CoM_star; dx_CoM_star];

        A_ds = [
            ((y_CoM - del_y_CoM_star*x_CoM)*(L0_ds - (x_CoM^2 + y_CoM^2)^(1/2)))/((x_CoM^2 + y_CoM^2)^(1/2)*(m_M + m_swLeg + m_swFoot)), (y_CoM*(L0_ds/(y_CoM^2 + (foot_prev - x_CoM)^2)^(1/2) - 1))/(m_M + m_swLeg + m_swFoot) + (del_y_CoM_star*(foot_prev - x_CoM)*(L0_ds/(y_CoM^2 + (foot_prev - x_CoM)^2)^(1/2) - 1))/(m_M + m_swLeg + m_swFoot)
            (x_CoM*(L0_ds/(x_CoM^2 + y_CoM^2)^(1/2) - 1))/(m_M + m_swLeg + m_swFoot),                                                                                                        -((foot_prev - x_CoM)*(L0_ds/(y_CoM^2 + (foot_prev - x_CoM)^2)^(1/2) - 1))/(m_M + m_swLeg + m_swFoot)];

        K_ds = [
            del2_y_CoM_star*dx_CoM^2 - K_p_ds*(y_CoM - y_CoM_star) - K_d_ds*(dy_CoM - del_y_CoM_star*dx_CoM) - (k0_ds*y_CoM*(L0_ds/(x_CoM^2 + y_CoM^2)^(1/2) - 1) - gravi*(m_M + m_swLeg + m_swFoot) + k0_ds*y_CoM*(L0_ds/(y_CoM^2 + (foot_prev - x_CoM)^2)^(1/2) - 1))/(m_M + m_swLeg + m_swFoot) - (del_y_CoM_star*(k0_ds*(foot_prev - x_CoM)*(L0_ds/(y_CoM^2 + (foot_prev - x_CoM)^2)^(1/2) - 1) - k0_ds*x_CoM*(L0_ds/(x_CoM^2 + y_CoM^2)^(1/2) - 1)))/(m_M + m_swLeg + m_swFoot);
            del_dx_CoM_star*dx_CoM - K_v_ds*(dx_CoM - dx_CoM_star) + (k0_ds*(foot_prev - x_CoM)*(L0_ds/(y_CoM^2 + (foot_prev - x_CoM)^2)^(1/2) - 1) - k0_ds*x_CoM*(L0_ds/(x_CoM^2 + y_CoM^2)^(1/2) - 1))/(m_M + m_swLeg + m_swFoot)];

        % % regularization terms
        % eps_ds = 5e-5;
        % eps_4 = eps_ds/det(A_ds);
        % eps_5 = eps_ds/det(A_ds);
        %
        % E_ds = [1/(eps_4 + 1), 0; 0, 1/(eps_5 + 1)];
        %
        % U_ds = E_ds*(A_ds^-1)*K_ds;

        det_A_ds = det(A_ds);

        % if abs(det_A_ds) >= 1e-9
        if abs(det_A_ds) >= 4e-9
            U_ds = (A_ds^-1)*K_ds;
            u4 = U_ds(1);
            u5 = U_ds(2);
        else
            u4 = 0;
            u5 = 0;
        end
    end

end

U = [u1; u2; u3; u4; u5];

% clipped = max(min(x, upper), lower);
var_stiff_bound_cst = 0.5;
upper = (1 + var_stiff_bound_cst);
lower = (var_stiff_bound_cst - 1);
U = [
    max(min(u1, k0_ss*upper), k0_ss*lower);
    max(min(u2, k_swLeg*upper), k_swLeg*lower);
    max(min(u3, k_swFoot*upper), k_swFoot*lower);
    max(min(u4, k0_ds*upper), k0_ds*lower);
    max(min(u5, k0_ds*upper), k0_ds*lower)];
